simulink library "snn_champions_lib"  (R2026a)
settings: Solver=VariableStepAuto
(part 5 of 24)

== matlab function snn_champions_lib/Donatello_ACC_IIDM_M/IIDM_CTRL ==
  data: s input; accel output; v input; dv input; v_l input
function accel = IIDM_CTRL(s, v, dv, v_l)
%#codegen
% SP4-M-FSM #2a - Donatello + ACC-IIDM con le 5 divisioni sequenziate su UNA divide() condivisa.
%  UNA sola chiamata a fsm_div in tutto il sorgente, dentro uno stato della FSM -> HDL Coder genera
%  UN divisore, riusato in 5 cicli. `kdiv` e' STATO, non indice di loop: un `for k=1:5` verrebbe
%  SROTOLATO dal codegen -> 5 divisori (giusto nel model acc_iidm_fsm, LETALE qui).
%  Nessun blocco accanto alla chart -> niente conversione MATLAB-to-dataflow -> tanh fixed NATIVA:
%  e' cio' che ha ucciso #1 (blocco Divide esterno) -- HDL_PHASE §9.
%  La matematica NON e' qui: sta in iidm_prep/iidm_nd/iidm_use/iidm_final, le STESSE del model
%  acc_iidm_fsm (G2: dmax=0 su 60000 control-step). Qui c'e' solo l'orchestrazione.
%
%  UNO STADIO PER CICLO (misurato: la prima versione faceva decode+prep in un ciclo e nd+div+use in
%  un altro -> path critico 701 livelli, Fmax 2,85 MHz, timing non chiuso). Il time-mux della FSM
%  taglia l'AREA; l'Fmax la da' il REGISTRO fra gli stadi: ogni fase fa UNA cosa e latcha il
%  risultato, cosi' il path piu' lungo e' al massimo quello di uno stadio (la divisione).
  Tt = snn_types('fixed', 13);
  Ta = acc_types('fixed');
  xn = local_normalize(s, v, dv, v_l, Tt);
  % alf/vlp (stato del filtro OU) vivono QUI, nel top-level: HDL Coder vieta i persistent in una
  % funzione non-entry-point chiamata in un condizionale, e iidm_prep e' chiamata in due rami.
  persistent pv xprev started acc phase kdiv st alf vlp rawl numl denl ql thl dA dR dQ dB dsq dkbit dns sX sR sQ sk sabv dkv dfrv blv ouv dsv acbl dadj qaf qbf ds0 ddel
  if isempty(started)
    pv = fi(zeros(5,1), 1, 21, 13);
    xprev = xn; started = true;
    acc = cast(0, 'like', Ta.out);
    phase = uint8(0); kdiv = uint8(1);
    alf = cast(0, 'like', Ta.acc); vlp = cast(v_l, 'like', Ta.st);
    % [R9] ouv: il TIPO viene dall'espressione dentro iidm_prep_a, non da una dichiarazione
    [ouv, alf, vlp] = iidm_prep_a(v_l, true, alf, vlp);
    % `pv(:)` (fi) e NON zeros(5,1) (double): due tipi diversi di `p` darebbero DUE specializzazioni
    % di iidm_prep, in silenzio.
    % [R2] stato della radice sequenziale: X radicando (consumato 2 bit per passo), R resto,
    % Q radice parziale, sk contatore di passi (STATO: un for verrebbe srotolato -> 10 radici).
    sX = fi(0, 0, sqrt_seq_nb()*2, 0); sR = fi(0, 0, sqrt_seq_nb()+2, 0);
    sQ = fi(0, 0, sqrt_seq_nb(), 0);   sk = uint8(0);
    % Il TIPO di sabv lo da' sqrt_seq_fin, non una costante scritta a mano: una sola definizione
    % (su un argomento nullo e' un reinterpretcast di una costante -> zero hardware).
    sabv = sqrt_seq_fin(sQ);
    % [R4] stato fra le due meta' del decode. I tipi sono quelli delle uscite di decode_a: se
    % sbagliassi, il codegen fallisce RUMOROSAMENTE (conflitto di tipo su persistent), non in silenzio.
    dkv = zeros(5,1,'int32'); dfrv = fi(zeros(5,1), 1, 16, 14);
    dsv = fi(zeros(5,1), 1, 16, 14);   % tipo Ts, lo stesso dichiarato in decode_b
    ds0 = fi(zeros(5,1), 1, 16, 14); ddel = fi(zeros(5,1), 1, 16, 14);   % [R17] tipo Ts
    dadj = fi(zeros(5,1), 1, 18, 13);   % tipo Tadj, lo stesso dichiarato in decode_a1
    [qaf, qbf] = iidm_ab(pv(:));   % [R14] tipi dedotti da iidm_ab (T.par)
    [st, alf, vlp] = iidm_prep(s, v, dv, v_l, pv(:), true, alf, vlp, sabv);
    rawl = fi(zeros(5,1), 1, 21, 13);   % latch del readout SNN: spezza il path SNN -> decode
    numl = cast(0, 'like', Ta.acc); denl = cast(1, 'like', Ta.acc); ql = cast(0, 'like', Ta.acc);
    % [IIDM #2] stato della ricorrenza: A dividendo residuo, R resto, Q quoziente, B divisore,
    % dsq segno, dkbit contatore di bit (STATO: un for verrebbe srotolato -> 27 divisori).
    dA = fi(0, 0, div_seq_nb(), 0); dQ = fi(0, 0, div_seq_nb(), 0);
    dR = fi(0, 0, 20, 0); dB = fi(0, 0, 20, 0);
    dsq = false; dkbit = uint8(0); dns = int8(0);
    % thl col TIPO NATIVO di tanh (NON cast a Ta.acc: butterebbe i bit frazionari del tanh prima
    % del prodotto con bf -> bug §2.1). Il tipo lo da' tanh stesso su un argomento di tipo Ta.acc.
    thl = tanh(cast(0, 'like', Ta.acc));
    % [R6] blv DOPO st e thl: il suo TIPO viene dall'espressione, non da una dichiarazione a mano
    % (cosi' non posso sbagliare la larghezza). Ordine obbligato: iidm_final_a li usa entrambi.
    blv = iidm_final_a(st, thl);
    acbl = iidm_final_b(st, blv);   % stesso principio: TIPO dedotto dall'espressione
    go = true;
  else
    go = any(xn ~= xprev);             % edge-triggered: 1 campione = 1 inferenza (§3.1.4)
  end
  xprev = xn;
  [raw, valid] = snn_b2_fsm(xn, go);
  if phase == 1                        % [R4] DECODE-A: indice di tabella + frazione
    dadj = decode_a1(rawl);
    phase = uint8(20);
  elseif phase == 20                   % [R12] DECODE-A2: scala, indice di tabella e frazione
    [dkv, dfrv] = decode_a2(dadj, 64);
    phase = uint8(12);
  elseif phase == 12                   % [R4] DECODE-B: interpolazione -> i 5 parametri IIDM
    [ds0, ddel] = decode_b1(dkv, 64);
    phase = uint8(23);
  elseif phase == 23                   % [R17] DECODE-B2: interpolazione lineare s0 + frac*del
    dsv = decode_b2(ds0, ddel, dfrv);
    phase = uint8(18);
  elseif phase == 18                   % [R10] DECODE-C: scalatura finale -> i 5 parametri
    pv = decode_c(dsv);
    phase = uint8(10);
  elseif phase == 10                   % [R2] SQRT-INIT: il radicando af*bf entra nella ricorrenza
    [qaf, qbf] = iidm_ab(pv(:));
    phase = uint8(21);
  elseif phase == 21                   % [R14] SQRT-PRE: il prodotto af*bf entra nella ricorrenza
    sX = sqrt_seq_setup(iidm_sabx_mul(qaf, qbf));
    sR(:) = 0; sQ(:) = 0; sk = uint8(sqrt_seq_nb());
    phase = uint8(11);
  elseif phase == 11                   % [R2] SQRT-STEP: 2 bit di radicando per ciclo, 10 cicli
    [sX, sR, sQ] = sqrt_seq_step(sX, sR, sQ);
    sk = sk - uint8(1);
    if sk == uint8(0)
      sabv = sqrt_seq_fin(sQ);         % SQRT-FIN: tipizzazione finale (reinterpretcast, zero HW)
      phase = uint8(2);
    end
  elseif phase == 2                    % PREP (un ciclo a se': guardie, filtro OU; la sqrt arriva fatta)
    [ouv, alf, vlp] = iidm_prep_a(v_l, false, alf, vlp);   % 1 volta per control-step (§5)
    phase = uint8(17);
  elseif phase == 17                   % [R9] OU-B: il passo esponenziale del filtro
    alf = iidm_prep_a2(ouv, alf);
    phase = uint8(16);
  elseif phase == 16                   % [R8] PREP-B: cast + costruzione dello struct
    st = iidm_prep_b(s, v, dv, v_l, pv(:), alf, sabv);
    kdiv = uint8(1); phase = uint8(3);
  elseif phase == 3                    % ND: SOLO gli operandi della divisione k
    [numl, denl] = iidm_nd(kdiv, st);
    phase = uint8(4);
  elseif phase == 4                    % DIV-INIT: magnitudini + segno (div_seq_setup)
    [dA, dB, dsq] = div_seq_setup(numl, denl);
    dR(:) = 0; dQ(:) = 0; dkbit = uint8(div_seq_nb());
    dns = int8(0);
    if numl > 0
      dns = int8(1);
    elseif numl < 0
      dns = int8(-1);
    end
    phase = uint8(8);
  elseif phase == 8                    % DIV-STEP: UN bit di quoziente per ciclo
    [dA, dR, dQ] = div_seq_step(dA, dR, dQ, dB);
    dkbit = dkbit - uint8(1);
    if dkbit == uint8(0)
      phase = uint8(9);
    end
  elseif phase == 9                    % DIV-FIN: segno + saturazione -> ql
    ql(:) = div_seq_fin(dQ, dsq, dB == 0, dns);
    phase = uint8(5);
  elseif phase == 5                    % [R5] USE-A: SOLO i quadrati (k=2: q^2, k=3: z e z^2)
    st = iidm_use_a(kdiv, ql, st);
    phase = uint8(15);
  elseif phase == 15                   % [R7] USE-M: il secondo quadrato (k=2: uu^2)
    st = iidm_use_m(kdiv, st);
    phase = uint8(22);
  elseif phase == 22                   % [R16] USE-M2: secondo quadrato (k=2) / sottrazione (k=3)
    st = iidm_use_m2(kdiv, st);
    phase = uint8(13);
  elseif phase == 13                   % [R5] USE-B: prodotti e selezioni
    st = iidm_use_b(kdiv, ql, st);
    if kdiv >= 5
      phase = uint8(6);
    else
      kdiv = kdiv + 1; phase = uint8(3);
    end
  elseif phase == 6                    % TANH: stadio a se' -- era il PATH CRITICO (237 liv, 7,35 MHz)
    thl(:) = iidm_tanh(st);
    phase = uint8(7);
  elseif phase == 7                    % [R6] FINAL-A: a_cah + bf*th (il prodotto col tanh)
    blv = iidm_final_a(st, thl);
    phase = uint8(14);
  elseif phase == 14                   % [R6] FINAL-B: blend + clamp -> accel (tenuta fino al prossimo)
    acbl = iidm_final_b(st, blv);
    phase = uint8(19);
  elseif phase == 19                   % [R11] FINAL-C: cast + selezione ACC + clamp -> accel
    acc = iidm_final_c(st, acbl);
    phase = uint8(0);
  end
  if valid                             % [2d R1] latch DOPO la catena: rawl e' un vero registro
    rawl(:) = raw;                     %   -> readout (pR_idx->raw) e decode (rawl->pv) DISACCOPPIATI
    phase = uint8(1);
  end
  accel = acc;
end

function xn = local_normalize(s, v, dv, v_l, T)
%LOCAL_NORMALIZE  fisico -> xn (fixed). Nel deployato la normalize gira in SW float e all'HDL
%  arriva gia' xn (HDL_PHASE §3.1); qui sta nel blocco per avere I/O fisico.
%  RECIPROCI a Q?.30 (NON Q?.20): verificato che con Q?.20 l'arrotondamento di xn devia di 1 LSB
%  dal path float ~1 volta su 25 step -> uno spike flippa -> i params divergono. Con Q?.30 e
%  ingressi con >=20 bit frazionari, xn e' IDENTICO al riferimento float (0 diff).
  invS   = fi(0.0066666666666666671, 1, 34, 30);
  invV   = fi(0.025000000000000001, 1, 34, 30);
  inv2DV = fi(0.025000000000000001, 1, 34, 30);
  invVL  = fi(0.025000000000000001, 1, 34, 30);
  DVc    = fi(20, 1, 24, 13);   % 24-13-1 = 10 bit interi: DV=20 ci sta
                                     % (con Q5.13/18bit saturerebbe a ~16 -> clamp sbagliato)
  d = dv;                            % clamp a +-DV. NB: d(:) = ... per NON cambiare il tipo di d
  if d >  DVc, d(:) =  DVc; end      %     (codegen: una variabile non puo' cambiare tipo, HDL_PHASE §9)
  if d < -DVc, d(:) = -DVc; end
  xn = cast(zeros(4,1), 'like', T.V);
  xn(1) = cast(s * invS, 'like', T.V);
  xn(2) = cast(v * invV, 'like', T.V);
  xn(3) = cast((d + DVc) * inv2DV, 'like', T.V);
  xn(4) = cast(v_l * invVL, 'like', T.V);
end

% ====================================================================================
% Funzioni locali INLINATE dai sorgenti veri (build_hdl_variants le legge a build-time).
% Le funzioni locali hanno precedenza sul path => il blocco e' SELF-CONTAINED.
% NON modificarle qui: si rigenerano con build_hdl_variants.
% ====================================================================================

function W = b2_rom_active() %#codegen
%B2_ROM_ACTIVE  Pesi del champion attivo (baked). GENERATO da gen_b2_rom('Donatello').
  W.fc = fi([1 1 -0.25 1;0.125 0.5 -0.0625 1;1 -1 1 0.125;1 0.125 0.5 -0.125;1 0.5 -0.0625 0.5;-0.0625 0.25 0 1;0 0.5 0.5 0.25;1 -0.25 2 -0.0625;1 0.125 -0.25 0.5;0.25 1 0.125 -0.25;0.25 -0.25 0.5 1;0.5 -0.5 0.5 0.25;1 0.25 -0.125 0.5;-1 1 0.25 0.5;1 0.5 1 -0.25;0.5 -0.25 0.5 0.0625;0.25 -0.25 1 -0.5;-0.5 -0.5 1 0.25;2 0 -0.25 0;-0.5 0.5 0.5 1;-0.125 -0.25 1 0;1 0.125 1 -0.5;-0.0625 1 0.5 0.125;1 1 -0.25 -0.125;2 0.5 0.5 -0.25;-0.125 0.5 0.25 -0.25;1 0.125 -0.0625 0.25;-0.5 -0.25 1 0.5;1 -0.125 0.125 0.5;1 -0.0625 0.5 0.25;1 0.5 1 0.125;0.125 0.25 0.5 0], 1, 16, 13);
  W.U = fi([0 0 -0.0625 -0.0625 -0.0625 0 0 0 -0.0625 0 0 0 0.0625 0 -0.125 0;-0.0625 0 -0.0625 0 0 0 0 0 0 0 -0.0625 0 0 0.0625 0 0;0.0625 -0.0625 -0.0625 0 -0.0625 -0.0625 0 0 0.0625 0 0.0625 0 0 0 0 0;0.0625 -0.0625 0 0 0 0 -0.0625 0 0 -0.0625 0.0625 -0.0625 0 -0.0625 0 -0.0625;0.0625 -0.0625 0 0 0 0 0.0625 0 0 0 0 -0.0625 0.0625 0 -0.0625 0;0 0.0625 0.0625 -0.0625 0.0625 0 0 0 0.0625 0.0625 0 0.0625 0 0 0 0;-0.0625 0.0625 0.0625 -0.0625 0 0 -0.0625 0.0625 0.0625 0.0625 0 0 -0.0625 0 0 0.0625;0 0 0.0625 0.0625 0 0 0 0 -0.0625 -0.0625 0 0 0 0 -0.0625 0;0 0 0 0 0.0625 -0.0625 0 0 -0.0625 -0.0625 -0.0625 0 0 0 0.0625 0;0 0 0 0 0.0625 0 0 0 0.0625 -0.0625 0 0.0625 0 0 0 0.0625;0 0 0 0 0 0 0 -0.0625 0 0 -0.0625 0 0 0 0 0.0625;0 0.0625 0 0.0625 0 0 0 0.0625 0 -0.0625 0 -0.0625 0.0625 0 0 0;-0.0625 0.0625 0 0 0 0 -0.0625 0 0.0625 0 -0.0625 0 0 0 0 0.125;0 0 0 0 0 0.0625 -0.0625 -0.0625 0 0.0625 0 0 0.0625 0.0625 0.0625 0;0.0625 0.0625 -0.0625 0 0 -0.0625 -0.0625 0 0 0 -0.0625 0 -0.0625 0 0 0;0.0625 0 0 0 -0.0625 -0.0625 -0.0625 0.0625 -0.0625 -0.0625 0 0.0625 0 0 0 0.0625;-0.0625 0 0 0 0.125 0.0625 -0.0625 -0.0625 0 0 0 0 -0.0625 0 -0.0625 0;0.0625 -0.0625 0 0.0625 0 -0.125 0 -0.0625 0 0 0.0625 -0.0625 0.0625 0 -0.0625 -0.0625;-0.0625 0 -0.0625 0.0625 -0.0625 0 -0.0625 0.0625 0.0625 -0.0625 0 0 -0.0625 0 0 -0.0625;0.0625 0.125 0 -0.0625 0 0 0 0 0.0625 0 0.0625 0.0625 0 0 -0.0625 0;0 -0.0625 0 0 -0.125 -0.0625 0 0.0625 -0.0625 -0.0625 0.0625 0 0.0625 -0.0625 -0.0625 -0.0625;0 0 0 0 -0.0625 0 0.0625 -0.0625 0 -0.0625 0.0625 0 0.0625 0 0 0;-0.0625 0.125 0 0 0 -0.0625 0 0 -0.0625 0.0625 0 0 0 0 0.0625 0;0 0 0 0 0 0 0 0 -0.0625 0 0.0625 0.125 0 0.0625 0 0.0625;0 -0.0625 0.0625 0 0 -0.0625 0 0 -0.0625 0 0 0.0625 0.0625 0 0 0;-0.0625 0 0 -0.125 0.0625 0.0625 0 0 0 0.0625 -0.0625 0.0625 -0.0625 0.0625 0.0625 0;0.0625 -0.0625 0 0 0 0 0.0625 0 -0.0625 0 0 0 0 0 0 0.0625;0 0 0 0.125 0 0 0 0.0625 -0.0625 0 0.0625 -0.0625 0 0.0625 0 0;0 0.0625 0.0625 0 0 0.0625 -0.0625 0 0 0.0625 0 0 -0.0625 0 0.0625 0.125;0 0.0625 0.0625 0.0625 0.0625 0.0625 0 0 0 0.0625 -0.0625 0.0625 -0.0625 0 0 0;0 0 0.0625 0 0 0.0625 -0.0625 -0.0625 0.0625 0.0625 -0.0625 0.125 0.0625 0 0 0;0 0 -0.0625 0.0625 0.0625 0 0 0.125 0 0.0625 0.0625 0.0625 0 -0.0625 0.0625 0], 1, 16, 13);
  W.Vr = fi([0 -0.125 -0.0625 -0.0625 0 0 -0.0625 -0.0625 0 -0.0625 -0.0625 0 0 0 -0.0625 -0.0625 0 0 0.0625 0 0 -0.125 0 0.0625 0 0 -0.0625 0 0 0 0 0;0.0625 0.0625 0 0 0 0 0.0625 0 0 0.0625 0.0625 0 0 0 0 0.0625 0 -0.0625 0 0.0625 0 0 0.0625 0 0.0625 0 0 0.125 -0.0625 0.125 0 0;0 0.0625 0 0.0625 0 0 -0.0625 0 0 0 0 0 0 0.0625 0 0 0.0625 0 0.0625 0 0 0.0625 0.0625 0 -0.0625 -0.0625 0 0 0 0.0625 0 0.0625;0 -0.0625 -0.0625 0 0 0 0 -0.0625 0 0 0.0625 0.0625 0 0 0 0.0625 0.0625 0 -0.0625 -0.0625 -0.0625 -0.0625 0.0625 0 0 0 0 0 0.0625 -0.0625 -0.0625 0;0 0 0.0625 0 -0.0625 0.0625 0.0625 0.0625 0 0 0.0625 0 0.0625 0.0625 0.0625 0 0.0625 0 0.0625 0 0.0625 0 0 0.0625 0.0625 0 0.125 0 0 0.0625 0.0625 0;0 0.0625 -0.125 0 0 0 0 0 0 -0.0625 -0.0625 0 0 0.0625 0.125 0.0625 0 0.0625 -0.0625 0.0625 0.0625 0 0.0625 -0.0625 0 -0.0625 0 0 0 0.0625 0 0;0 -0.0625 -0.0625 0 0 -0.0625 0 -0.0625 0 0 -0.0625 -0.0625 -0.0625 0.0625 -0.0625 0 0 -0.0625 0.0625 -0.125 -0.0625 0 -0.0625 -0.0625 -0.0625 0 0 -0.125 -0.0625 0 0 -0.0625;0 0 -0.0625 -0.0625 0.0625 0 -0.0625 0 -0.0625 0 0.0625 -0.0625 0.0625 0.0625 0.0625 0 0 0 0 -0.0625 0 -0.0625 0 0 0 0 -0.0625 -0.0625 0 0 0 0;-0.0625 0.0625 0 0.0625 0 0.0625 -0.0625 0 0.0625 0 0.0625 0 0 0.0625 0 0 0 0 0.0625 -0.0625 0.0625 0 0.0625 0 0 0.125 0.0625 0.0625 0.0625 0.0625 0 0;0.0625 0.0625 0 0.0625 0.0625 0.0625 0.0625 0.0625 0.0625 0 0.0625 0 0.0625 0.0625 0 -0.0625 0.0625 0 0.0625 0.0625 0 0.0625 0.0625 0 0.0625 0.0625 0 0 0 0 0 0;0 -0.0625 -0.0625 0 -0.0625 0 0 0 0 0 -0.0625 -0.125 -0.0625 -0.0625 0 -0.0625 -0.0625 0 0 -0.0625 -0.0625 0 0 0 0 -0.0625 0 -0.0625 0 0 -0.0625 0;0 0 0 0.0625 0 0 0.0625 0 0 0 0 0 0.0625 0 0 0.125 -0.0625 0 0.0625 0.0625 0 0 0.0625 0.0625 0 0.0625 0.0625 0 0 0 0 0;-0.0625 0 0 0 0.0625 0.0625 0 -0.0625 -0.0625 -0.0625 -0.0625 0 0 -0.0625 0 -0.0625 0 0 0 -0.0625 0 -0.0625 0 0 -0.0625 -0.0625 0 0 -0.0625 0 0.0625 0;0.0625 0 0 0.0625 0 0 0 -0.0625 0 0.0625 0 -0.0625 0 0.0625 0.0625 0 0.0625 0.0625 0 0.0625 0 0 0 0.0625 0.0625 0 0 0.125 0 0 0.0625 -0.0625;0.0625 0 0 0.0625 0 0.0625 0 0 0 0.0625 -0.0625 -0.0625 0 0.125 0 0 0 0 -0.0625 0 0.0625 0 0.0625 -0.0625 0.0625 0 0 0 0 0 0.0625 0;0 0 0 0.0625 0 0.0625 0 0.0625 0 0 0.0625 0.0625 0 0 0 0.0625 -0.0625 0 0.0625 0.0625 0.0625 0 0 0.0625 0.125 0 0 0 0 0 0.0625 0], 1, 19, 13);
  W.Wout = fi([-0.25 -0.125 -0.0625 -0.25 -0.25 0.25 0.25 -0.5 0.125 0.125 0.5 0.25 0.5 -0.125 0.25 0.25 -0.5 -0.25 0.0625 0.25 -0.25 0.0625 0 0.125 -0.25 0.25 0.25 -0.25 0 0 0.125 0.5;0.125 -0.125 0.25 -0.25 -0.125 0 -0.25 0 -0.25 0 0 0 -0.5 -0.5 0.125 0.25 -0.5 0.125 -0.25 0 0.25 0.25 -0.25 0.25 0.25 0 0.5 -0.25 -0.125 -0.25 0.0625 0.0625;0 -0.25 -0.25 0.125 -0.5 -0.0625 0 -0.125 0.125 0 0.25 -0.0625 -0.25 0.25 0.0625 -0.125 -0.25 0.125 -0.5 0.125 0.25 -0.5 -0.25 -0.25 0.25 0.25 0 0.5 -0.125 -0.5 0.125 0.125;0.5 0 0.25 0.25 0.25 -0.5 0.25 -0.25 0.5 0 -0.5 0.125 -0.0625 -0.5 -0.125 0.0625 0.25 -0.125 0.25 0.0625 0 0.0625 -0.25 -0.25 -0.125 -0.5 -0.25 0 -0.25 -0.125 -0.0625 -0.0625;-0.25 0 -0.0625 0.0625 0 -0.25 -0.125 -0.0625 -0.25 0 -0.0625 0.125 0.0625 0.25 -0.0625 -0.25 0.125 -0.25 -0.0625 -0.125 -0.25 -0.125 0.25 0.25 0.0625 0.25 -0.5 0.0625 0.25 0.25 -0.25 0.125], 1, 16, 13);
  W.bth = fi([1.4830578565597534;1.4914478063583374;1.4758200645446777;1.4738426208496094;1.4738566875457764;1.5251744985580444;1.5266332626342773;1.4767427444458008;1.4758551120758057;1.5250141620635986;1.5258395671844482;1.5129754543304443;1.5257152318954468;1.5249043703079224;1.5155367851257324;1.5183815956115723;1.5177655220031738;1.4894863367080688;1.4749715328216553;1.5253423452377319;1.4770052433013916;1.4827579259872437;1.5239431858062744;1.5230189561843872;1.4776254892349243;1.5125672817230225;1.5243701934814453;1.4934873580932617;1.5239229202270508;1.5202276706695557;1.5248651504516602;1.5149734020233154], 1, 19, 13);
  W.tj = fi([0.49987733364105225;0.49987733364105225;0.49987733364105225;0.49987733364105225;0.49987733364105225;0.49987733364105225;0.49987733364105225;0.49987733364105225;0.49987733364105225;0.49987733364105225;0.49987733364105225;0.49987733364105225;0.49987733364105225;0.49987733364105225;0.49987733364105225;0.49987733364105225;0.49987733364105225;0.49987733364105225;0.49987733364105225;0.49987733364105225;0.49987733364105225;0.49987733364105225;0.49987733364105225;0.49987733364105225;0.49987733364105225;0.49987733364105225;0.49987733364105225;0.49987733364105225;0.49987733364105225;0.49987733364105225;0.49987733364105225;0.49987733364105225], 1, 19, 13);
  W.delays = [3 5 1 2;2 4 4 4;2 4 0 4;5 0 5 5;1 2 2 2;4 1 4 2;0 4 0 1;0 1 0 1;2 2 1 3;1 2 5 2;0 5 1 2;0 5 3 1;2 0 0 4;2 2 3 4;4 4 5 0;4 5 0 2;0 4 4 3;5 5 4 2;4 5 4 2;3 0 3 1;3 2 0 4;0 4 2 0;5 4 5 2;4 4 3 3;5 3 4 5;2 2 3 1;3 3 5 3;1 3 0 3;1 0 3 2;2 3 4 4;2 4 5 0;1 2 4 0];
  W.sh = 3;
  W.invS = fi(0.0066666666666666671, 1, 24, 20);
  W.invV = fi(0.025000000000000001, 1, 24, 20);
  W.invVL = fi(0.025000000000000001, 1, 24, 20);
  W.inv2DV = fi(0.025000000000000001, 1, 24, 20);
  W.DV = fi(20, 1, 20, 13);
end


function T = snn_types(dt, nfrac)
%SNN_TYPES Prototipi di tipo per il core type-parametrizzato.
%  dt = 'double' (parita' vs golden) | 'fixed' (HDL, Qm.n).
%  nfrac (opz., default 5) = bit frazionari del path fixed; i bit INTERI restano
%  fissi (range invariato), varia solo la risoluzione -> per tarare i word-length
%  col ginocchio errore/risorse (run_fixed_sweep). nfrac=5 == config storica.
  if nargin < 2, nfrac = 5; end
  switch dt
    case 'double'
      z = double([]);
      T = struct('V', z, 'fatigue', z, 'acc', z, 'accw', z, 'raw', z, 'w', z);
    case 'fixed'
      f = nfrac;
      T = struct( ...
        'V',       fi([], true, 6 + f, f), ...    % Q5.f  (int 5)
        'fatigue', fi([], true, 4 + f, f), ...    % Q3.f  (int 3)
        'acc',     fi([], true, 6 + f, f), ...    % accumulatore I_input Q5.f (int 5: un tap di delay arriva a ~8)
        'accw',    fi([], true, 13 + f, f + 4), ...% accumulatore LARGO Q8.(f+4): +4 frac per shift po2 esatti
        'raw',     fi([], true, 8 + f, f), ...    % readout LI Q7.f (int 7)
        'w',       fi([], true, 3 + f, f));       % pesi po2 Q2.f (esatti per f>=5)
    otherwise
      error('snn_types:dt', 'dt deve essere ''double'' o ''fixed''');
  end
end


function [raw, valid] = snn_b2_fsm(xn, start) %#codegen
%SNN_B2_FSM  [B2] SNN Donatello time-multiplexato (1 neurone/clock) con hdl.RAM.
%  Mirror BIT-EXACT dell'aritmetica di snn_core, serializzato: V/fatigue in hdl.RAM,
%  pesi in ROM (coder.const), pipeline a 2 stadi per la latenza RAM (read->compute->write,
%  1 sola chiamata RAM/ciclo). Streaming: start=1 -> nuova control-step; valid=1 -> raw pronto.
  W = coder.const(b2_rom_active());
  T = snn_types('fixed', 13);
  hidden = 32; nt = 10; rnk = coder.const(size(W.U, 2)); out = 5; sh = W.sh;

  persistent Vram fatram xbuf xnreg t_lr t_lr_nxt V_LI wacc ...
             tickc rc written phase ...
             pR_valid pR_idx pCx_valid pCx_idx pCx_xsel pCx_Vread pCx_fat ...
             pCm_valid pCm_idx pCm_Iip pCm_recip pCm_Vread pCm_fat ...
             pCa_valid pCa_idx pCa_reci pCa_Ii pCa_Vread pCa_fat ...
             pC1_valid pC1_idx pC1_Ii pC1_reci pC1_Vread pC1_fat ...
             pC2i_valid pC2i_idx pC2i_Vi pC2i_eth pC2i_fat ...
             pC2a_valid pC2a_idx pC2a_nCV pC2a_sib pC2a_fat ...
             pC_valid pC_idx pC_V pC_fat rawreg inited
  if isempty(inited)
    Vram   = hdl.RAM('RAMType', 'Dual port');
    fatram = hdl.RAM('RAMType', 'Dual port');
    xbuf   = cast(zeros(4, 6), 'like', T.V);
    xnreg  = cast(zeros(4, 1), 'like', T.V);
    t_lr     = cast(zeros(rnk, 1), 'like', T.acc);
    t_lr_nxt = cast(zeros(rnk, 1), 'like', T.acc);
    V_LI = cast(zeros(out, 1), 'like', T.raw);
    wacc = cast(zeros(out, 1), 'like', T.raw);
    tickc = uint8(0); rc = uint8(0); written = uint8(0); phase = uint8(0);
    pR_valid = false; pR_idx = uint8(0);
    pCx_valid = false; pCx_idx = uint8(0);
    pCx_xsel = cast(zeros(4, 1), 'like', T.V);
    pCx_Vread = cast(0, 'like', T.V); pCx_fat = cast(0, 'like', T.fatigue);
    pCm_valid = false; pCm_idx = uint8(0);
    pCm_Iip = cast(zeros(4, 1), 'like', T.accw); pCm_recip = cast(zeros(rnk, 1), 'like', T.accw);
    pCm_Vread = cast(0, 'like', T.V); pCm_fat = cast(0, 'like', T.fatigue);
    pCa_valid = false; pCa_idx = uint8(0);
    pCa_reci = cast(zeros(rnk/4, 1), 'like', T.accw);   % rnk/4 somme parziali (dopo 2 livelli d'albero)
    pCa_Ii = cast(0, 'like', T.accw);
    pCa_Vread = cast(0, 'like', T.V); pCa_fat = cast(0, 'like', T.fatigue);
    pC1_valid = false; pC1_idx = uint8(0);
    pC1_Ii = cast(0, 'like', T.accw); pC1_reci = cast(0, 'like', T.accw);
    pC1_Vread = cast(0, 'like', T.V); pC1_fat = cast(0, 'like', T.fatigue);
    % [2d R8] prototipi dei tipi LARGHI di Vi/eth (l'addizione fixed li allarga oltre T.V): servono per
    % registrarli fra C2i (Vi/eth) e C2a (soglia/nC_V) senza conflitto di tipo in codegen.
    zV = cast(0, 'like', T.V); zA = cast(0, 'like', T.accw); zF = cast(0, 'like', T.fatigue);
    Vi0  = cast(zV - bitsra(zV, sh), 'like', T.V) + (zA + zA);
    eth0 = cast(zV, 'like', T.V) + cast(max(zF, zF), 'like', T.V);
    pC2i_valid = false; pC2i_idx = uint8(0);
    pC2i_Vi = cast(0, 'like', Vi0); pC2i_eth = cast(0, 'like', eth0);
    pC2i_fat = cast(0, 'like', T.fatigue);
    pC2a_valid = false; pC2a_idx = uint8(0);
    pC2a_nCV = cast(0, 'like', T.V); pC2a_sib = cast(0, 'like', T.V);
    pC2a_fat = cast(0, 'like', T.fatigue);
    pC_valid = false; pC_idx = uint8(0);
    pC_V = cast(0, 'like', T.V); pC_fat = cast(0, 'like', T.fatigue);
    rawreg = cast(zeros(out, 1), 'like', T.raw);
    inited = true;
  end

  valid = false;
  raw = rawreg;

  % ---------- helper x_buf: shift + inserimento xnreg (inizio tick) ----------
  % (fatto inline dove serve)

  if phase == uint8(0)
    % IDLE: su start latcha xn, fa lo shift del tick 0, avvia la pipeline
    if start
      xnreg = xn;
      xbuf(:, 2:6) = xbuf(:, 1:5); xbuf(:, 1) = xnreg;   % tick 0 shift+insert
      tickc = uint8(0); rc = uint8(0); written = uint8(0);
      wacc = cast(zeros(out, 1), 'like', T.raw);
      pR_valid = false; pC_valid = false;
      phase = uint8(1);
    end
    % passo RAM idle (mantiene coerenza)
    [~, ~] = Vram(cast(0,'like',T.V), uint8(0), false, uint8(0));
    [~, ~] = fatram(cast(0,'like',T.fatigue), uint8(0), false, uint8(0));
    return;
  end

  % ---------- FASE 1: RUN (pipeline 2-stadi, 1 chiamata RAM/ciclo) ----------
  % indirizzo di lettura per questo ciclo (neurone rc, se ancora da leggere)
  if rc < uint8(hidden), rdAddr = rc; else, rdAddr = uint8(0); end

  % UNA chiamata RAM: scrive il risultato dello stadio C (pC), legge rdAddr
  [~, Vread]   = Vram(pC_V,   pC_idx, pC_valid, rdAddr);
  [~, fatread] = fatram(pC_fat, pC_idx, pC_valid, rdAddr);
  if pC_valid
    written = written + uint8(1);
  end

  % --- STADIO Cx (mux xbuf: seleziona i 4 ingressi ritardati): dal neurone pR ---
  % [2d R9] separo il mux a indice variabile xbuf(j,col) dal DSP mult: Cx registra i 4 valori selezionati
  % (xsel), Cm fa solo i moltiplicatori dai valori registrati -> il mult (~4,6ns) resta l'unico op del suo path.
  nCx_valid = false; nCx_idx = uint8(0);
  nCx_xsel = cast(zeros(4, 1), 'like', T.V);
  nCx_Vread = cast(0, 'like', T.V); nCx_fat = cast(0, 'like', T.fatigue);
  if pR_valid
    i = double(pR_idx) + 1;
    for j = 1:4
      col = double(W.delays(i, j)) + 1;
      nCx_xsel(j) = xbuf(j, col);
    end
    nCx_Vread = Vread; nCx_fat = fatread;
    nCx_valid = true; nCx_idx = pR_idx;
  end

  % --- STADIO Cm (MAC: 16 prodotti reci + 4 prodotti Ii, REGISTRATI): dagli ingressi mux registrati pCx ---
  % [2d R6] isolo i moltiplicatori: Cm calcola e REGISTRA i prodotti (uscite DSP), Ca fa gli alberi dai
  % prodotti registrati -> il DSP mult (~4,6ns) esce dal path degli alberi (mappato sul registro P del DSP48).
  % Bit-exact: stessi prodotti, solo registrati.
  nCm_valid = false; nCm_idx = uint8(0);
  nCm_Iip = cast(zeros(4, 1), 'like', T.accw);
  nCm_recip = cast(zeros(rnk, 1), 'like', T.accw);
  nCm_Vread = cast(0, 'like', T.V); nCm_fat = cast(0, 'like', T.fatigue);
  if pCx_valid
    i = double(pCx_idx) + 1;
    for j = 1:4
      nCm_Iip(j) = cast(cast(W.fc(i, j), 'like', T.w) * pCx_xsel(j), 'like', T.accw);
    end
    for r = 1:rnk
      nCm_recip(r) = cast(cast(W.U(i, r), 'like', T.w) * t_lr(r), 'like', T.accw);
    end
    nCm_Vread = pCx_Vread; nCm_fat = pCx_fat;
    nCm_valid = true; nCm_idx = pCx_idx;
  end

  % --- STADIO Ca (alberi: Ii 4->1, reci L1-L2 16->4): dai prodotti registrati pCm ---
  kmid = coder.const(rnk / 4);                    % rnk=16 -> 4 parziali dopo 2 livelli
  nCa_valid = false; nCa_idx = uint8(0);
  nCa_reci = cast(zeros(kmid, 1), 'like', T.accw);
  nCa_Ii = cast(0, 'like', T.accw);
  nCa_Vread = cast(0, 'like', T.V); nCa_fat = cast(0, 'like', T.fatigue);
  if pCm_valid
    % Ii ad albero (4->2->1) dai prodotti registrati
    Ii_p = pCm_Iip;
    Ii_p(1) = cast(Ii_p(1) + Ii_p(2), 'like', T.accw);
    Ii_p(2) = cast(Ii_p(3) + Ii_p(4), 'like', T.accw);
    nCa_Ii  = cast(Ii_p(1) + Ii_p(2), 'like', T.accw);
    % reci: primi 2 livelli d'albero (16->4) dai prodotti registrati
    reci_p = pCm_recip;
    lvsz_a = coder.const(round(rnk ./ 2 .^ (1:2)));   % rnk=16 -> [8 4]
    for lev = 1:2
      for q = 1:lvsz_a(lev)
        reci_p(q) = cast(reci_p(2*q - 1) + reci_p(2*q), 'like', T.accw);
      end
    end
    nCa_reci = reci_p(1:kmid);            % rnk/4 somme parziali (T.accw)
    nCa_Vread = pCm_Vread; nCa_fat = pCm_fat;
    nCa_valid = true; nCa_idx = pCm_idx;
  end

  % --- STADIO C1 (SECONDA meta' dell'albero reci): dal registro pCa ---
  nC1_valid = false; nC1_idx = uint8(0);
  nC1_Ii = cast(0, 'like', T.accw); nC1_reci = cast(0, 'like', T.accw);
  nC1_Vread = cast(0, 'like', T.V); nC1_fat = cast(0, 'like', T.fatigue);
  if pCa_valid
    reci_p2 = pCa_reci;                  % kmid parziali
    lvsz_b = coder.const(round(kmid ./ 2 .^ (1:log2(kmid))));   % kmid=4 -> [2 1]
    for lev = 1:numel(lvsz_b)
      for q = 1:lvsz_b(lev)
        reci_p2(q) = cast(reci_p2(2*q - 1) + reci_p2(2*q), 'like', T.accw);
      end
    end
    nC1_reci = reci_p2(1);
    nC1_Ii = pCa_Ii; nC1_Vread = pCa_Vread; nC1_fat = pCa_fat;   % Vi/soglia -> C2 (tipi larghi restano locali)
    nC1_valid = true; nC1_idx = pCa_idx;
  end

  % --- STADIO C2i (calcola Vi ed eth, tipi larghi 28-bit): dal registro pC1 ---
  % [2d R8] separo Vi/eth (catena di add 28-bit, era il collo in C2a-R7) dalla soglia/nC_V: C2i li produce
  % e REGISTRA (tipi larghi via prototipo Vi0/eth0 in init; init nel corpo via 'like' pC2i_*). Bit-exact.
  nC2i_valid = false; nC2i_idx = uint8(0);
  nC2i_Vi = cast(0, 'like', pC2i_Vi); nC2i_eth = cast(0, 'like', pC2i_eth);
  nC2i_fat = cast(0, 'like', T.fatigue);
  if pC1_valid
    i2 = double(pC1_idx) + 1;
    nC2i_Vi  = cast(pC1_Vread - bitsra(pC1_Vread, sh), 'like', T.V) + (pC1_Ii + pC1_reci);
    nC2i_eth = cast(W.bth(i2), 'like', T.V) + cast(max(pC1_fat, cast(0,'like',T.fatigue)), 'like', T.V);
    nC2i_fat = pC1_fat;
    nC2i_valid = true; nC2i_idx = pC1_idx;
  end

  % --- STADIO C2a (soglia + nC_V + accumulo readout): dal registro pC2i ---
  nC2a_valid = false; nC2a_idx = uint8(0);
  nC2a_nCV = cast(0, 'like', T.V); nC2a_sib = cast(0, 'like', T.V);
  nC2a_fat = cast(0, 'like', T.fatigue);
  if pC2i_valid
    i2  = double(pC2i_idx) + 1;
    si  = pC2i_Vi >= pC2i_eth;
    sib = cast(si, 'like', T.V);
    nC2a_nCV = cast(pC2i_Vi - sib * pC2i_eth, 'like', T.V);
    nC2a_sib = sib; nC2a_fat = pC2i_fat;
    nC2a_valid = true; nC2a_idx = pC2i_idx;
    if si
      for o = 1:out
        wacc(o) = cast(wacc(o) + W.Wout(o, i2), 'like', T.raw);
      end
      for r = 1:rnk
        t_lr_nxt(r) = cast(t_lr_nxt(r) + cast(W.Vr(r, i2), 'like', T.acc), 'like', T.acc);
      end
    end
  end

  % --- STADIO C2b (nC_fat = leaky(fat) + sib*tj): dal registro pC2a; nC_V passa attraverso ---
  nC_valid = false; nC_idx = uint8(0);
  nC_V = cast(0, 'like', T.V); nC_fat = cast(0, 'like', T.fatigue);
  if pC2a_valid
    i3 = double(pC2a_idx) + 1;
    nC_fat = cast(cast(pC2a_fat - bitsra(pC2a_fat, sh), 'like', T.fatigue) + pC2a_sib * cast(W.tj(i3), 'like', T.V), 'like', T.fatigue);
    nC_V   = pC2a_nCV;
    nC_valid = true; nC_idx = pC2a_idx;
  end

  % --- STADIO R (read schedule): programma la lettura del neurone rc ---
  nR_valid = false; nR_idx = uint8(0);
  if rc < uint8(hidden)
    nR_valid = true; nR_idx = rc;
    rc = rc + uint8(1);
  end

  % avanza i registri pipeline (R -> Cm -> Ca -> C1 -> C2 -> write)
  pR_valid = nR_valid; pR_idx = nR_idx;
  pCx_valid = nCx_valid; pCx_idx = nCx_idx; pCx_xsel = nCx_xsel; pCx_Vread = nCx_Vread; pCx_fat = nCx_fat;
  pCm_valid = nCm_valid; pCm_idx = nCm_idx; pCm_Iip = nCm_Iip; pCm_recip = nCm_recip; pCm_Vread = nCm_Vread; pCm_fat = nCm_fat;
  pCa_valid = nCa_valid; pCa_idx = nCa_idx; pCa_reci = nCa_reci; pCa_Ii = nCa_Ii; pCa_Vread = nCa_Vread; pCa_fat = nCa_fat;
  pC1_valid = nC1_valid; pC1_idx = nC1_idx; pC1_Ii = nC1_Ii; pC1_reci = nC1_reci; pC1_Vread = nC1_Vread; pC1_fat = nC1_fat;
  pC2i_valid = nC2i_valid; pC2i_idx = nC2i_idx; pC2i_Vi = nC2i_Vi; pC2i_eth = nC2i_eth; pC2i_fat = nC2i_fat;
  pC2a_valid = nC2a_valid; pC2a_idx = nC2a_idx; pC2a_nCV = nC2a_nCV; pC2a_sib = nC2a_sib; pC2a_fat = nC2a_fat;
  pC_valid = nC_valid; pC_idx = nC_idx; pC_V = nC_V; pC_fat = nC_fat;

  % --- fine tick: tutti i 32 neuroni scritti ---
  if written >= uint8(hidden)
    V_LI = cast(cast(V_LI - bitsra(V_LI, 3), 'like', T.raw) + wacc, 'like', T.raw);
    wacc = cast(zeros(out, 1), 'like', T.raw);
    t_lr = t_lr_nxt;
    t_lr_nxt = cast(zeros(rnk, 1), 'like', T.acc);
    written = uint8(0); rc = uint8(0);
    pR_valid = false; pCx_valid = false; pCm_valid = false; pCa_valid = false; pC1_valid = false; pC2i_valid = false; pC2a_valid = false; pC_valid = false;
    if tickc >= uint8(nt - 1)
      rawreg = V_LI; raw = V_LI; valid = true;
      phase = uint8(0); tickc = uint8(0);
    else
      tickc = tickc + uint8(1);
      xbuf(:, 2:6) = xbuf(:, 1:5); xbuf(:, 1) = xnreg;   % shift+insert per il tick successivo
    end
  end
end

% ---- ROM pesi del champion attivo: in b2_rom_active.m (baked, GENERATO da gen_b2_rom(name)) ----


function p = snn_decode_lut(raw, N) %#codegen
%SNN_DECODE_LUT  Decode Donatello con sigmoide via LUT a N punti su [-8,8) + interp lineare.
%  Generalizza snn_decode_hdl (N=256). N = coder.const, potenza di 2 (scala indice = N/16).
%  Costanti Donatello baked (lo sweep e' Donatello-only). Bit-identico a snn_decode_hdl per N=256.
%
%  ⚠️ SINGLE SOURCE (R4, 2026-07-19): il corpo e' ora la composizione di decode_a + decode_b, che sono
%  le DUE FASI che la chart esegue in due clock distinti -- il decode era il collo (pv_3, 31 livelli:
%  quattro moltiplicatori in serie piu' la lettura di tabella, tutto in un clock).
%  Composte qui in una chiamata sola perche' (a) i chiamanti non cambiano (snn_top_b2, le varianti
%  Donatello_LUT16..512) e (b) i cancelli provano ESATTAMENTE il codice che gira in hardware, non un
%  suo gemello. Il taglio e' fra `frac` e la lettura di `sgtab`: espressioni invariate, solo separate.
  [k, frac] = decode_a(raw, N);
  sv        = decode_b(k, frac, N);
  p         = decode_c(sv);   % [R10] scalatura finale in una fase a se'
end


function [k, frac] = decode_a(raw, N) %#codegen
%DECODE_A  [R4/R12] Prima meta' del decode: dal readout grezzo all'INDICE di tabella + frazione.
%
%  ⚠️ SINGLE SOURCE: composizione di decode_a1 (normalizzazione) e decode_a2 (scala/indice/frazione),
%  che la chart esegue in DUE clock -- i due moltiplicatori erano in serie (collo a 57,5 MHz).
%  Composta qui per i chiamanti funzionali (snn_decode_lut) e perche' i cancelli provino il codice vero.
%
%  ⚠️ NON si time-multiplexano i 5 parametri (restano srotolati): sarebbe un'ottimizzazione di AREA, e
%  di area ce n'e' in abbondanza. Serve solo profondita'.
  adjv        = decode_a1(raw);
  [k, frac]   = decode_a2(adjv, N);
end


function adjv = decode_a1(raw) %#codegen
%DECODE_A1  [R12] Prima parte del decode: normalizzazione (raw - offset)*invtau.
%  Separata da decode_a2 perche' i due moltiplicatori (invtau e scale) erano in serie nello stesso
%  clock -- era il collo a 57,5 MHz (dfrv, 18 livelli). `adj` ha il tipo Tadj GIA' DICHIARATO
%  nell'originale, quindi qui non si stringe nulla (nessun rischio §2.1).
%  Espressione VERBATIM da snn_decode_lut.
  Traw  = numerictype(1,21,13); Tadj = numerictype(1,18,13); Titau = numerictype(1,18,16);
  offset = coder.const(fi([-0.40404 -0.39012 1.7718 2.6884 -0.95578].', Traw));
  invtau = coder.const(fi([0.1 1/3 0.1 1/3 1/3].', Titau));
  adjv = fi(zeros(5,1), Tadj);
  for i = 1:5
    adjv(i) = fi((raw(i) - offset(i)) * invtau(i), Tadj);
  end
end


function [k, frac] = decode_a2(adjv, N) %#codegen
%DECODE_A2  [R12] Seconda parte: scala su [0,N), indice di tabella e frazione.
%  Espressioni VERBATIM da snn_decode_lut, con `adj` gia' calcolato da decode_a1.
  Tadj = numerictype(1,18,13); Ts = numerictype(1,16,14); Tsc = numerictype(0,23,13);
  scale = coder.const(N / 16);                                    % punti per unita' su [-8,8)
  Tsm   = numerictype(0, 8, 0);                                   % moltiplicatore scala (<=32)
  k    = zeros(5, 1, 'int32');
  frac = fi(zeros(5,1), Ts);
  for i = 1:5
    scaled = fi((adjv(i) + fi(8, Tadj)) * fi(scale, Tsm), Tsc);    % (adj+8)*scale in [0,N)
    ki = int32(floor(scaled));
    if ki < int32(0),     ki = int32(0);     end
    if ki > int32(N - 2), ki = int32(N - 2); end
    k(i)    = ki;
    frac(i) = fi(scaled - fi(double(ki), Tsc), Ts);
  end
end


function sv = decode_b(k, frac, N) %#codegen
%DECODE_B  [R4/R10/R17] Seconda fase del decode: tabella + interpolazione lineare -> s.
%  ⚠️ SINGLE SOURCE: composizione di decode_b1 (letture + differenza) e decode_b2 (interpolazione), che
%  la chart esegue in DUE clock. Composta qui per i chiamanti funzionali e per i cancelli.
  [s0v, delv] = decode_b1(k, N);
  sv          = decode_b2(s0v, delv, frac);
end


function [s0v, delv] = decode_b1(k, N) %#codegen
%DECODE_B1  [R17] Letture della tabella + differenza: s0 = sgtab(k), del = sgtab(k+1) - sgtab(k).
%  Separata da decode_b2 perche' letture, sottrazione, moltiplicazione e somma erano tutte nello stesso
%  clock -- era il collo a 77,6 MHz (dsv, 14 livelli). Espressioni VERBATIM da snn_decode_lut.
  Ts    = numerictype(1,16,14);
  scale = coder.const(N / 16);
  sgtab = coder.const(fi(1 ./ (1 + exp(-(-8 + (0:N-1) / scale))), Ts));  % 1xN
  s0v  = fi(zeros(5,1), Ts);
  delv = fi(zeros(5,1), Ts);
  for i = 1:5
    s0 = sgtab(k(i) + 1); s1 = sgtab(k(i) + 2);
    s0v(i)  = s0;
    delv(i) = fi(s1 - s0, Ts);
  end
end


function sv = decode_b2(s0v, delv, frac) %#codegen
%DECODE_B2  [R17] Interpolazione lineare: s = s0 + frac*del. Espressione VERBATIM da snn_decode_lut.
  Ts = numerictype(1,16,14);
  sv = fi(zeros(5,1), Ts);
  for i = 1:5
    sv(i) = fi(s0v(i) + frac(i) * delv(i), Ts);
  end
end


function p = decode_c(sv) %#codegen
%DECODE_C  Scalatura finale -> i 5 parametri. [R10] fase a se' nel controllore.
%  [A3] Ora e' la COMPOSIZIONE di decode_c1 (i prodotti, a precisione piena) + decode_c2 (somma
%  dell'offset + cast). Composta qui perche' (a) i chiamanti non cambiano e (b) i cancelli provano
%  ESATTAMENTE il codice che gira in hardware, non un suo gemello.
%  La chart nella variante `p6` chiama le due meta' in due fasi distinte: e' li' che il taglio serve,
%  perche' separa i DSP dalla catena di CARRY4 che domina il path critico.
  pr = decode_c1(sv);
  p  = decode_c2(pr);
end


function pr = decode_c1(sv) %#codegen
%DECODE_C1  [A3] Prima meta' di decode_c: i SOLI PRODOTTI hilo.*sv.
%  Taglio dentro l'operazione, non fra le operazioni: il collo di Donatello e' `lo + hilo*sv`, dove i
%  DSP fanno la moltiplicazione ma la somma finisce in fabric come catena di 15 CARRY4 in serie
%  (misurato: 24,307 ns = logica 15,490 + routing 8,817, 23 livelli).
%  Registrare il prodotto separa DSP e addizionatore in due clock.
%
%  ⚠️ LARGHEZZA PIENA: il prodotto NON va stretto qui. Stringere un parziale prima dell'uso e' il bug
%  §2.1 di questo progetto — cambierebbe la matematica. Il tipo si lascia DEDURRE dall'espressione.
  Tp   = numerictype(1,21,13);
  hilo = coder.const(fi([37 2 4 2.2 2.5].', Tp));
  pr   = hilo .* sv;                  % tipo dedotto = precisione piena
end


function p = decode_c2(pr) %#codegen
%DECODE_C2  [A3] Seconda meta' di decode_c: somma dell'offset + cast finale ai 5 parametri.
%  Riceve il prodotto a PRECISIONE PIENA da decode_c1 (registrato) e fa `lo + pr`, poi il cast a Q8.13.
%  Aritmetica IDENTICA a decode_c: stesso ordine, stesso singolo cast finale -> bit-exact per
%  costruzione. Ma "per costruzione" non e' un cancello: lo prova run_block_traj_test (dmax=0).
  Tp = numerictype(1,21,13);
  lo = coder.const(fi([8 0.5 1 0.3 0.5].', Tp));
  p  = fi(zeros(5,1), Tp);
  for i = 1:5
    p(i) = fi(lo(i) + pr(i), Tp);
  end
end


function T = acc_types(dt, nfrac, recipN)
%ACC_TYPES  Prototipi di tipo per `acc_iidm_open` type-parametrizzato (modello: snn_types.m).
%  dt = 'double' (riferimento algoritmico + plant cf_plant_lib) | 'fixed' (blocco HDL-ready).
%  nfrac (opz.) = bit frazionari del path fixed; i bit INTERI restano FISSI (il range non cambia),
%  varia solo la risoluzione -> e' la manopola dello sweep (run_acc_fixed_sweep), esattamente come
%  snn_types/run_fixed_sweep fanno per la rete.
%
%  I bit INTERI sono dimensionati con DUE criteri diversi, perche' i limiti hanno natura diversa --
%  applicare a tutti la stessa regola sarebbe misurare la cosa sbagliata:
%
%  (A) limitati dall'OSSERVAZIONE -> margine >= 2x sul massimo misurato (il dataset non e' il mondo).
%      Range misurati su 60 traiettorie x 1000 step coi parametri veri stimati dalla rete (spec SP3 §3):
%    st  : s, v, dv, v_l, s_safe, s_star         max misurato  465.77 -> int 10 (|x|<1024, 2.2x)
%    acc : v_free, a_z, a_iidm, a_cah, a_blend,
%          alf, a_l_bar, dd, z, dv^2/(2*s_safe)  min misurato -288.33 -> int 10 (|x|<1024, 3.6x)
%
%  (B) limitati da un CLAMP -> basta che il tipo copra il limite: non e' una stima, non puo' sforare.
%      Un margine di 1.4x su un limite CERTO vale piu' di 2x su un massimo osservato.
%    par : v0,T,s0,a,b   il decode li vincola a [param_lo, param_hi] = [8 .5 1 .3 .5]..[45 2.5 5 2.5 3]
%                        (sigmoide * range + lo: non puo' uscirne)   -> int  6 (|x|<64, 1.4x su 45)
%    out : accel         il codice la clampa a [-9, a], con a <= 2.5 -> int  4 (|x|<16, 1.8x su 9)
  % nfrac di DEFAULT = 8: il MINIMO che rispetta il budget DERIVATO. Misurato da run_acc_fixed_sweep
  % sul dataset INTERO (60 traj x 1000 step = 60.000 campioni, 2026-07-16, log sweep_nfrac8_60traj.log):
  %   budget  E_snn  (footprint in accel della quantizzazione GIA' accettata della rete):
  %                                   p99 = 0.272054   max = 1.48433  [m/s^2]
  %   nfrac=6 E_iidm  p99 = 0.324937  max = 1.78485  -> NON passa (l'IIDM diventerebbe la fonte
  %                                                     d'errore DOMINANTE, scavalcando la rete)
  %   nfrac=8 E_iidm  p99 = 0.156047  max = 0.83368  -> passa, margine ~1.75x su entrambi
  % ⚠️ Passa STRETTO: un dry-run su 2 traiettorie dava ~6x di margine, il dataset intero dice 1.75x.
  %    Le code stanno solo nel campione completo -> non tarare questo numero su pochi casi.
  if nargin < 2, nfrac = 8; end
  % recipN: strategia di divisione del path fixed. 0 = divide() digit-recurrence (SP3, combinatorio
  % profondo). >0 = reciproco a LUT a recipN punti + moltiplica (SP4 variante L). Vive nei tipi cosi'
  % la scelta e' coder.const e single-source. Default 0 = comportamento SP3 invariato.
  if nargin < 3, recipN = 0; end
  switch dt
    case 'double'
      z = double([]);
      T = struct('st', z, 'par', z, 'acc', z, 'out', z);
      T.recipN = 0;
    case 'fixed'
      f = nfrac;
      % La fimath fa parte del TIPO, non e' una decorazione locale. Due ragioni, entrambe misurate:
      %  1) RoundingMethod 'Zero' e' l'UNICA forma di divisione che HDL Coder genera per tipi signed
      %     ('Floor' vale solo per unsigned, 'Nearest' viene rifiutata) -- spec SP3 §2;
      %  2) attaccarla qui evita che una `setfimath` locale la cambi su una variabile gia' assegnata:
      %     il codegen rifiuta anche il cambio di FIMATH, non solo di tipo -- "Properties of fimath
      %     object must match. Property 'RoundMode' is 'nearest' ... but 'fix'". Mettendola nel
      %     prototipo, ogni cast(x,'like',T.*) la porta con se' e tutto combacia per costruzione.
      % Prodotti e somme a precisione FISSA: senza, i word-length crescerebbero a ogni operazione.
      FM = fimath('RoundingMethod', 'Zero', 'OverflowAction', 'Saturate', ...
                  'ProductMode', 'SpecifyPrecision', ...
                  'ProductWordLength', 11 + f, 'ProductFractionLength', f, ...
                  'SumMode', 'SpecifyPrecision', ...
                  'SumWordLength', 11 + f, 'SumFractionLength', f);
      % Prototipi con valore 0 e NON `fi([])`: un campo VUOTO e' "empty-typed" e HDL Coder lo rifiuta
      % quando lo struct dei tipi attraversa piu' funzioni -- "Struct in expression 'acc_types(''fixed'')'
      % has an empty-typed field. This is not supported for MATLAB-to-dataflow conversion" (SP4-M-FSM:
      % le funzioni-fase iidm_prep/nd/use/final). Come PROTOTIPO e' equivalente: `cast(x,'like',T.*)` usa
      % solo numerictype+fimath, che qui sono identici -> nessun cambiamento numerico (lo provano
      % run_plant_parity, run_block_acciidm_test e G2, tutti ri-eseguiti dopo questa modifica).
      T = struct( ...
        'st',  fi(0, true, 11 + f, f, FM), ...   % Q10.f
        'par', fi(0, true,  7 + f, f, FM), ...   % Q6.f
        'acc', fi(0, true, 11 + f, f, FM), ...   % Q10.f
        'out', fi(0, true,  5 + f, f, FM));      % Q4.f
      T.recipN = recipN;
    otherwise
      error('acc_types:dt', 'dt deve essere ''double'' o ''fixed''');
  end
end


function q = fsm_div(num, den) %#codegen
%FSM_DIV  [SP4-M-FSM] La divisione della forma FSM: UNICA implementazione. FIXED-ONLY.
%  E' la STESSA divisione di acc_div con recipN=0, cioe' SP3: divide(numerictype(T.acc), num, den) con
%  la fimath di acc_types (RoundingMethod 'Zero', l'unica che HDL Coder genera per signed - SP3 §2).
%
%  ⚠️ `T` COSTRUITO DENTRO e non ricevuto come argomento: HDL Coder rifiuta uno struct di prototipi che
%     attraversa le funzioni -- "Struct in expression 'T' has an empty-typed field. This is not supported
%     for MATLAB-to-dataflow conversion" (i prototipi di acc_types sono fi([],...), campi VUOTI).
%     Chiamata qui dentro con argomento letterale, acc_types e' coder.const e viene ripiegata.
%     Conseguenza accettata: la forma FSM e' fixed-only. Il riferimento DOUBLE resta acc_iidm_open
%     (type-parametrico, invariato) -- lo prova run_plant_parity.
%
%  Nella chart del blocco M le 5 divisioni a divisore VARIABILE non passano di qui: sono sostituite
%  dall'handshake verso HDLMathLib/Divide, che G1 ha provato BIT-IDENTICO a questa divide() su 300.000
%  coppie reali (dmax=0). La divisione a divisore COSTANTE (DT del filtro OU) resta qui anche nel blocco:
%  per una costante HDL Coder ripiega un moltiplicatore shallow, non e' un collo di profondita'.
  T = acc_types('fixed');
  q = divide(numerictype(T.acc), num, den);
end


function [st, alf, vlp] = iidm_prep(s, v, dv, v_l, p, rst, alf, vlp, sabin) %#codegen
%IIDM_PREP  [SP4-M-FSM] Fase 0 della FSM: guardie, cast, filtro OU, sab, s_safe -> stato `st`.
%
%  ⚠️ `sabin` (R2, 2026-07-19) = sqrt(af*bf) GIA' CALCOLATA dal chiamante, non piu' qui dentro.
%  Motivo: la radice era il COLLO (17,5 MHz, tutti i 400 path peggiori finivano su st_sab) e per
%  sequenzializzarla serve piu' di un clock -- impossibile dentro una funzione-fase che gira in UNO.
%  Chi chiama la calcola come sa: il model in un colpo (`sqrt_seq`), la chart in 10 stadi con la STESSA
%  ricorrenza (sqrt_seq_step). Vedi iidm_sabx per l'ingresso, che e' a fonte unica.
%  Matematica VERBATIM da acc_iidm_open (righe 24-57): stesse espressioni, stessi cast, stesso ordine.
%
%  UNICA implementazione, chiamata SIA dal model (acc_iidm_fsm, per G2 sul dataset) SIA dalla chart del
%  blocco `Donatello_ACC_IIDM_M` -> la matematica non puo' divergere fra i due (e' il buco §2.1 che
%  costo' l'82,4% dei control-step su snn_b2_fsm: due implementazioni della stessa matematica).
%
%  `st` esce con TUTTI i campi gia' tipizzati (i parziali a zero): da qui in poi i campi non cambiano
%  piu' tipo -- gli aggiornamenti usano `st.campo(:) = ...` (HDL_PHASE §9: una variabile non puo'
%  cambiare ne' tipo ne' fimath).
%
%  ⚠️ Una chiamata per CONTROL-STEP (DT=0.1): il filtro OU stima a_l da Δv_l/DT. Chiamarla a ogni clock
%     farebbe vedere Δv_l=0 per 340 campioni su 341 -> a_l~0, in silenzio (spec SP2 §5).
  % T COSTRUITO DENTRO (non ricevuto): HDL Coder rifiuta uno struct di prototipi che attraversa le
  % funzioni -- "Struct in expression 'T' has an empty-typed field ... MATLAB-to-dataflow conversion"
  % (acc_types usa fi([],...), campi VUOTI). Con argomento letterale e' coder.const -> ripiegata.
%
%  ⚠️ SINGLE SOURCE (R8, 2026-07-19): composizione di iidm_prep_a (SOLO il filtro OU) e
%  iidm_prep_b (cast + costruzione dello struct), che la chart esegue in DUE clock -- il filtro OU
%  era il collo (alf -> a_l_bar, gradini 8 e 9 della scala). G2 prova sui 60000 control-step che il
%  taglio e' bit-neutro.
  [d, alf, vlp] = iidm_prep_a(v_l, rst, alf, vlp);   % R9: differenza finita
  alf           = iidm_prep_a2(d, alf);              % R9: passo esponenziale
  st         = iidm_prep_b(s, v, dv, v_l, p, alf, sabin);
end


function [d, alf, vlp] = iidm_prep_a(v_l, rst, alf, vlp) %#codegen
%IIDM_PREP_A  [R9] Prima meta' del filtro OU: la DIFFERENZA FINITA del leader, d = (lq - vlp)/DT.
%  `d` esce a LARGHEZZA PIENA e senza tipo dichiarato -- lo si lascia dedurre dall'espressione, come per
%  blv in R6: cosi' non si puo' sbagliare la larghezza, e stringerlo cambierebbe la matematica (§2.1).
%
%  ORDINE OBBLIGATO (verbatim da iidm_prep): d usa il vlp VECCHIO, e solo DOPO vlp viene aggiornato.
%  Con rst, vlp = v_l -> d = 0 e alf = 0: inizio traiettoria pulito.
  T = acc_types('fixed');
  DT = 0.1;
  if rst
    alf(:) = 0;
    vlp(:) = v_l;
  end
  lq = cast(v_l, 'like', T.st);
  % Moltiplicazione per 1/DT invece di divide(): vedi iidm_prep. Bit-identita' provata da G2.
  INV_DT = 1/DT;
  d   = (lq - vlp) * INV_DT;
  vlp = cast(lq, 'like', T.st);
end


function alf = iidm_prep_a2(d, alf) %#codegen
%IIDM_PREP_A2  [R9] Seconda meta' del filtro OU: il passo esponenziale.
%  Era il collo a 46,3 MHz (alf_7, 21 livelli): differenza finita e filtro stavano nello stesso clock.
%  Espressione VERBATIM da iidm_prep, con (lq-vlp)*INV_DT gia' calcolato in `d`.
  T = acc_types('fixed');
  DT = 0.1; ALPHA = exp(-DT/1.0);
  alf = cast(ALPHA*alf + (1-ALPHA)*d, 'like', T.acc);
end


function st = iidm_prep_b(s, v, dv, v_l, p, alf, sabin) %#codegen
%IIDM_PREP_B  [R8] Cast, guardie e costruzione dello stato `st`, a partire dall'`alf` GIA' aggiornato
%  da iidm_prep_a (registrato fra i due clock). Espressioni VERBATIM da iidm_prep.
  T = acc_types('fixed');
  v0 = max(p(1), 1e-3); T_ = max(p(2), 1e-3); s0 = p(3);   % a,b -> iidm_ab (servono anche a iidm_sabx)

  sq = cast(s,  'like', T.st);   vq = cast(v,   'like', T.st);
  dq = cast(dv, 'like', T.st);   lq = cast(v_l, 'like', T.st);   %#ok<NASGU>
  v0f = cast(v0, 'like', T.par); Tf_ = cast(T_, 'like', T.par); s0f = cast(s0, 'like', T.par);
  [af, bf] = iidm_ab(p);         % fonte unica, condivisa con iidm_sabx (l'ingresso della radice)

  sab    = cast(max(sabin, 1e-6), 'like', T.par);   % la radice arriva GIA' FATTA
  s_safe = cast(max(sq, 2.0), 'like', T.st);

  % Tipi PIENI dei quadrati (R5/R7): stringerli cambierebbe la matematica (bug §2.1).
  sq0 = cast(0, 'like', T.acc) * cast(0, 'like', T.acc);
  sq1 = sq0 * sq0;
  sq2 = 1 - sq0;
  vt0 = cast(0, 'like', T.st) * cast(0, 'like', T.par);   % [R15] tipo pieno di vq*Tf_     % [R13] tipo pieno di (1 - z^2): isolare la sottrazione dai prodotti

  st = struct( ...
    'vq',      vq, ...
    'dq',      dq, ...
    'v0f',     v0f, ...
    'Tf_',     Tf_, ...
    's0f',     s0f, ...
    'af',      af, ...
    'bf',      bf, ...
    'sab',     sab, ...
    's_safe',  s_safe, ...
    'a_l_bar', cast(min(alf, af), 'like', T.acc), ...
    's_star',  cast(0, 'like', T.st), ...
    'v_free',  cast(0, 'like', T.acc), ...
    'z',       cast(0, 'like', T.acc), ...
    'a_iidm',  cast(0, 'like', T.acc), ...
    'a_cah',   cast(0, 'like', T.acc), ...
    'dd',      cast(0, 'like', T.acc), ...
    'uu',      cast(0, 'like', sq0), ...
    'zz',      cast(0, 'like', sq0), ...
    'uu2',     cast(0, 'like', sq1), ...
    'w',       cast(0, 'like', sq2), ...
    'vt',      cast(0, 'like', vt0), ...
    'qm',      cast(0, 'like', T.acc));
end


function [num, den] = iidm_nd(k, st) %#codegen
%IIDM_ND  [SP4-M-FSM] (num,den) della divisione k, presi dallo stato `st`. UNICA implementazione: la
%  chiamano sia il model (acc_iidm_fsm) sia la chart del blocco M (che li manda al blocco Divide).
%
%  Le 5 divisioni a divisore VARIABILE (ordine = dipendenze: q3 dopo q1 via s_star; q5 dopo q3/q4 via
%  a_iidm/a_cah). Espressioni VERBATIM da acc_iidm_open (righe 56, 58, 59, 68, 70).
%
%  ENTRAMBI in T.acc: il cast e' LOSSLESS (la fimath di acc_types ha Product/SumMode SpecifyPrecision
%  a 11+f bit con f=8 -> ogni prodotto/somma e' GIA' Q10.8 = T.acc; e T.par Q6.8 ⊂ T.acc Q10.8, stessi
%  frazionari). Serve perche' (a) una variabile non puo' cambiare tipo fra i rami (§9) e (b) il blocco
%  Divide ha porte di tipo fisso. G1 ha provato la bit-identita' proprio su coppie in T.acc; G2 ri-verifica
%  end-to-end che il cast non muova un bit.
  T = acc_types('fixed');           % costruito DENTRO (vedi iidm_prep): HDL Coder rifiuta lo struct come arg
  num = cast(0, 'like', T.acc);
  den = cast(1, 'like', T.acc);
  if k == 1                                   % q1 = vq*dq / (2*sab)            -> s_star
    num(:) = st.vq * st.dq;
    den(:) = 2*st.sab;
  elseif k == 2                               % q2 = vq / v0f                   -> v_free
    num(:) = st.vq;
    den(:) = st.v0f;
  elseif k == 3                               % q3 = s_star / s_safe            -> z
    num(:) = st.s_star;
    den(:) = st.s_safe;
  elseif k == 4                               % q4 = max(dq,0)^2 / (2*s_safe)   -> a_cah
    num(:) = max(st.dq, 0)^2;
    den(:) = 2*st.s_safe + 1e-6;
  else                                        % q5 = (a_iidm-a_cah) / bf        -> dd
    num(:) = st.a_iidm - st.a_cah;
    den(:) = st.bf + 1e-6;
  end
end


function st = iidm_use(k, q, st) %#codegen
%IIDM_USE  [SP4-M-FSM] Consuma il quoziente q della divisione k e aggiorna lo stato `st`. UNICA
%  implementazione: la chiamano sia il model (acc_iidm_fsm) sia la chart del blocco M.
%
%  ⚠️ SINGLE SOURCE (R5, 2026-07-19): il corpo e' ora la composizione di iidm_use_a (i quadrati) e
%  iidm_use_b (prodotti e selezioni), che la chart esegue in DUE clock distinti -- k=2 e k=3 erano le
%  due catene piu' profonde della legge (quattro e due moltiplicatori in serie). Composte qui in una
%  chiamata sola: il model resta a un passo e G2 prova sui 60000 control-step che il taglio e' bit-neutro.
  st = iidm_use_a(k, q, st);
  st = iidm_use_m(k, st);      % [R7/R16] primi quadrati
  st = iidm_use_m2(k, st);     % [R16] secondo quadrato / sottrazione
  st = iidm_use_b(k, q, st);
end


function st = iidm_use_a(k, q, st) %#codegen
%IIDM_USE_A  [R5/R16] Prima fase del consumo del quoziente: SOLO i clamp (nessuna moltiplicazione).
%  La legge IIDM ha due catene lunghe, ora distribuite su QUATTRO fasi:
%    k=2  min -> ^2 -> ^2 -> *af      (v_free)
%    k=3  min -> ^2 -> (1-z^2) -> *   (a_iidm)
%  Qui sta solo il primo anello: il clamp. Era il collo a 72,9 MHz (st_uu: min e quadrato insieme).
  if k == 2
    st.qm(:) = min(q, 10);
  elseif k == 3
    st.z(:)  = min(q, 20);
  end
end


function st = iidm_use_m(k, st) %#codegen
%IIDM_USE_M  [R7] Fase di MEZZO del consumo del quoziente: il secondo quadrato di k=2.
%  st.v_free = af*(1 - min(q,10)^4) aveva ANCORA due moltiplicatori in serie dopo R5 (uu^2, poi *af):
%  era il collo a 42,6 MHz (st_v_free, 25 livelli). Qui si isola uu^2 dietro un registro.
%  Il campo `uu2` ha il tipo PIENO (~104 bit): costa registri, non moltiplicatori -- il prodotto
%  esisteva gia', si sta solo mettendo un registro DOPO di esso.
  if k == 1
    st.vt(:) = st.vq * st.Tf_;   % [R15] il prodotto esce dal clock di s_star
  elseif k == 2
    st.uu(:) = st.qm^2;          % [R16] primo quadrato (qm = min(q,10) da iidm_use_a)
  elseif k == 3
    st.zz(:) = st.z^2;           % [R16] quadrato di z
  end
end


function st = iidm_use_m2(k, st) %#codegen
%IIDM_USE_M2  [R16] Terza fase: il secondo quadrato di k=2 e la sottrazione di k=3.
%  Espressioni VERBATIM; i campi hanno il tipo PIENO del prodotto (vedi iidm_prep_b).
  if k == 2
    st.uu2(:) = st.uu^2;
  elseif k == 3
    st.w(:) = 1 - st.zz;
  end
end


function st = iidm_use_b(k, q, st) %#codegen
%IIDM_USE_B  [R5] Seconda meta': i prodotti e le selezioni, a partire dai quadrati gia' registrati.
%  Espressioni VERBATIM da iidm_use, con `min(q,10)^4` -> `st.uu^2` e `st.z^2` -> `st.zz`: identita'
%  garantita solo perche' uu/zz sono a LARGHEZZA PIENA (iidm_prep). Il cancello e' G2 sui 60000
%  control-step -- non si assume che le due forme coincidano, si prova.
  T = acc_types('fixed');
  if k == 1                                   % q1 -> s_star
    st.s_star(:) = st.s0f + max(st.vt + q, 0);   % [R15] vt = vq*Tf_ arriva da iidm_use_m

  elseif k == 2                               % q2 -> v_free
    st.v_free(:) = st.af*(1 - st.uu2);   % [R7] uu2 = uu^2 arriva da iidm_use_m

  elseif k == 3                               % q3 -> a_z / a_iidm (z e z^2 arrivano da iidm_use_a)
    below = (st.vq <= st.v0f);
    a_z = cast(st.af*st.w, 'like', T.acc);
    if st.z < 1
      if below, st.a_iidm(:) = st.v_free*st.w; else, st.a_iidm(:) = st.v_free; end
    else
      if below, st.a_iidm(:) = a_z;                   else, st.a_iidm(:) = st.v_free + a_z; end
    end

  elseif k == 4                               % q4 -> a_cah (+ clamp)
    st.a_cah(:) = st.a_l_bar - q;
    st.a_cah(:) = min(max(st.a_cah, -9), st.af);

  else                                        % q5 -> dd
    st.dd(:) = q;
  end
end


function th = iidm_tanh(st) %#codegen
%IIDM_TANH  [SP4-M-FSM · B2.0-2b] Stadio del tanh: th = tanh(st.dd), via LUT PIENA bit-exact.
%  Dopo lo Studio 2b (document/SP4_ACC_IIDM_FAST.md §Studio 2b): il `tanh` nativo di HDL Coder era il
%  collo combinatorio (198 livelli, 9,42 MHz standalone). `tanh_lut_full` lo MEMOIZZA (LUT 4096 su
%  [-8,8) + 2 costanti di saturazione) -> **dmax=0**, bit-identico al nativo (provato: probe_tanh_dmax
%  = 0 su 20000 control-step a livello accel), ma **8 livelli / 136 MHz standalone e 0 DSP**, ed e' piu'
%  PICCOLA del nativo (545 vs 2190 LUT). Nel controllore intero il tanh non e' piu' il collo (L2 ~10,58,
%  cappato da SNN->decode).
%
%  ⚠️ th resta sfix19_En17 (tipo nativo del tanh): NON castarlo a T.acc (En8) -> butterebbe i bit
%     frazionari prima del prodotto per bf in iidm_final (bug §2.1). La LUT emette gia' sfix19_En17.
%  Confronto delle 5 varianti (native/LUT/interp/poly/CORDIC): SP4_ACC_IIDM_FAST.md §Studio 2b.
%  `tanh_lut_full` e' inlinata nel chart da build_hdl_variants; la tabella la genera gen_tanh_lut().
  th = tanh_lut_full(st.dd);
end


function th = tanh_lut_full(dd) %#codegen
% [B2.0-2b A1] tanh via LUT PIENA bit-exact: memoizza tanh(fi(x,1,19,8)) su [-8,8),
%  saturazione oltre. th: sfix19_En17. GENERATO da gen_tanh_lut.m -- NON modificare a mano.
  persistent TBL
  if isempty(TBL)
    TBL = int32([ ...
      -131070
      -131070
      -131070
      -131070
      -131070
      -131070
      -131070
      -131070
      -131070
      -131070
      -131070
      -131070
      -131070
      -131070
      -131070
      -131070
      -131070
      -131070
      -131070
      -131070
      -131070
      -131070
      -131070
      -131070
      -131070
      -131070
      -131070
      -131070
      -131070
      -131070
      -131070
      -131070
      -131070
      -131070
      -131070
      -131070
      -131070
      -131070
      -131070
      -131070
      -131070
      -131070
      -131070
      -131070
      -131070
      -131070
      -131070
      -131070
      -131070
      -131070
      -131070
      -131070
      -131070
      -131070
      -131070
      -131070
      -131070
      -131070
      -131070
      -131070
      -131070
      -131070
      -131070
      -131070
      -131070
      -131070
      -131070
      -131070
      -131070
      -131070
      -131070
      -131070
      -131070
      -131070
      -131070
      -131070
      -131070
      -131070
      -131070
      -131070
      -131070
      -131070
      -131070
      -131070
      -131070
      -131070
      -131070
      -131070
      -131070
      -131070
      -131070
      -131070
      -131070
      -131070
      -131070
      -131070
      -131070
      -131070
      -131070
      -131070
      -131070
      -131070
      -131070
      -131070
      -131070
      -131070
      -131070
      -131070
      -131070
      -131070
      -131070
      -131070
      -131070
      -131070
      -131070
      -131070
      -131070
      -131070
      -131070
      -131070
      -131070
      -131070
      -131070
      -131070
      -131070
      -131070
      -131070
      -131070
      -131070
      -131070
      -131070
      -131070
      -131070
      -131070
      -131070
      -131070
      -131070
      -131070
      -131070
      -131070
      -131070
      -131070
      -131070
      -131070
      -131070
      -131070
      -131070
      -131070
      -131070
      -131070
      -131070
      -131070
      -131070
      -131070
      -131070
      -131070
      -131070
      -131070
      -131070
      -131070
      -131070
      -131070
      -131070
      -131070
      -131070
      -131070
      -131070
      -131070
      -131070
      -131070
      -131070
      -131070
      -131070
      -131070
      -131070
      -131070
      -131070
      -131070
      -131070
      -131070
      -131070
      -131070
      -131070
      -131070
      -131070
      -131070
      -131070
      -131070
      -131070
      -131070
      -131070
      -131070
      -131070
      -131070
      -131070
      -131070
      -131070
      -131070
      -131070
      -131070
      -131070
      -131070
      -131070
      -131070
      -131070
      -131070
      -131070
      -131070
      -131070
      -131070
      -131070
      -131070
      -131070
      -131070
      -131070
      -131070
      -131070
      -131070
      -131070
      -131070
      -131070
      -131070
      -131070
      -131070
      -131070
      -131070
      -131070
      -131070
      -131070
      -131070
      -131070
      -131070
      -131070
      -131070
      -131070
      -131070
      -131070
      -131070
      -131070
      -131070
      -131070
      -131070
      -131070
      -131070
      -131070
      -131070
      -131070
      -131070
      -131070
      -131070
      -131070
      -131070
      -131070
      -131070
      -131070
      -131070
      -131070
      -131070
      -131070
      -131070
      -131070
      -131070
      -131070
      -131070
      -131070
      -131070
      -131070
      -131070
      -131070
      -131070
      -131070
      -131070
      -131070
      -131070
      -131070
      -131070
      -131070
      -131070
      -131070
      -131070
      -131070
      -131070
      -131070
      -131070
      -131070
      -131070
      -131070
      -131070
      -131070
      -131070
      -131070
      -131070
      -131070
      -131070
      -131070
      -131070
      -131070
      -131070
      -131070
      -131070
      -131070
      -131070
      -131070
      -131070
      -131070
      -131070
      -131070
      -131070
      -131070
      -131070
      -131070
      -131070
      -131070
      -131070
      -131070
      -131070
      -131070
      -131070
      -131070
      -131070
      -131070
      -131070
      -131070
      -131070
      -131070
      -131070
      -131070
      -131070
      -131070
      -131070
      -131070
      -131070
      -131070
      -131070
      -131070
      -131070
      -131070
      -131070
      -131070
      -131070
      -131070
      -131070
      -131070
      -131070
      -131070
      -131070
      -131070
      -131070
      -131070
      -131070
      -131070
      -131070
      -131070
      -131070
      -131070
      -131070
      -131070
      -131070
      -131070
      -131070
      -131070
      -131070
      -131070
      -131070
      -131070
      -131070
      -131070
      -131070
      -131070
      -131070
      -131070
      -131070
      -131070
      -131070
      -131070
      -131070
      -131070
      -131070
      -131070
      -131070
      -131070
      -131070
      -131070
      -131070
      -131070
      -131070
      -131070
      -131070
      -131070
      -131070
      -131070
      -131070
      -131070
      -131070
      -131070
      -131070
      -131070
      -131070
      -131070
      -131070
      -131070
      -131070
      -131070
      -131070
      -131070
      -131070
      -131070
      -131070
      -131070
      -131070
      -131070
      -131070
      -131070
      -131070
      -131070
      -131070
      -131070
      -131070
      -131070
      -131070
      -131070
      -131070
      -131070
      -131070
      -131070
      -131070
      -131070
      -131070
      -131070
      -131070
      -131070
      -131070
      -131070
      -131070
      -131070
      -131070
      -131070
      -131070
      -131070
      -131070
      -131070
      -131070
      -131070
      -131070
      -131070
      -131070
      -131070
      -131070
      -131070
      -131070
      -131070
      -131070
      -131070
      -131070
      -131070
      -131070
      -131070
      -131070
      -131070
      -131070
      -131070
      -131070
      -131070
      -131070
      -131070
      -131070
      -131070
      -131070
      -131070
      -131070
      -131070
      -131070
      -131070
      -131070
      -131070
      -131070
      -131070
      -131070
      -131070
      -131070
      -131070
      -131070
      -131070
      -131070
      -131070
      -131070
      -131070
      -131070
      -131070
      -131070
      -131070
      -131070
      -131070
      -131070
      -131070
      -131070
      -131070
      -131070
      -131070
      -131070
      -131070
      -131070
      -131070
      -131070
      -131070
      -131070
      -131070
      -131070
      -131070
      -131070
      -131070
      -131070
      -131070
      -131070
      -131070
      -131070
      -131070
      -131070
      -131070
      -131070
      -131070
      -131070
      -131070
      -131070
      -131070
      -131070
      -131070
      -131070
      -131070
      -131070
      -131070
      -131070
      -131070
      -131070
      -131070
      -131070
      -131070
      -131070
      -131070
      -131070
      -131070
      -131070
      -131070
      -131070
      -131070
      -131070
      -131070
      -131070
      -131070
      -131070
      -131070
      -131070
      -131070
      -131070
      -131070
      -131070
      -131070
      -131070
      -131070
      -131070
      -131070
      -131070
      -131070
      -131070
      -131070
      -131070
      -131070
      -131070
      -131070
      -131070
      -131070
      -131070
      -131070
      -131070
      -131070
      -131070
      -131070
      -131070
      -131070
      -131070
      -131070
      -131070
      -131070
      -131070
      -131070
      -131070
      -131070
      -131070
      -131070
      -131070
      -131070
      -131070
      -131070
      -131070
      -131070
      -131070
      -131070
      -131070
      -131070
      -131070
      -131070
      -131070
      -131070
      -131070
      -131070
      -131070
      -131070
      -131070
      -131070
      -131070
      -131070
      -131070
      -131070
      -131070
      -131070
      -131070
      -131070
      -131070
      -131070
      -131070
      -131070
      -131070
      -131070
      -131070
      -131070
      -131070
      -131070
      -131070
      -131070
      -131070
      -131070
      -131070
      -131070
      -131070
      -131070
      -131070
      -131070
      -131070
      -131070
      -131070
      -131070
      -131070
      -131070
      -131070
      -131070
      -131070
      -131070
      -131070
      -131070
      -131070
      -131070
      -131070
      -131070
      -131070
      -131070
      -131070
      -131070
      -131070
      -131070
      -131070
      -131070
      -131070
      -131070
      -131070
      -131070
      -131070
      -131070
      -131070
      -131070
      -131070
      -131070
      -131070
      -131070
      -131070
      -131070
      -131070
      -131070
      -131070
      -131070
      -131070
      -131070
      -131070
      -131070
      -131070
      -131070
      -131070
      -131070
      -131070
      -131070
      -131070
      -131070
      -131070
      -131070
      -131070
      -131070
      -131070
      -131070
      -131070
      -131070
      -131070
      -131070
      -131070
      -131070
      -131070
      -131070
      -131070
      -131070
      -131070
      -131070
      -131070
      -131070
      -131070
      -131070
      -131070
      -131070
      -131070
      -131070
      -131070
      -131070
      -131070
      -131070
      -131070
      -131070
      -131070
      -131070
      -131070
      -131070
      -131070
      -131070
      -131070
      -131070
      -131070
      -131070
      -131070
      -131070
      -131070
      -131070
      -131070
      -131070
      -131070
      -131070
      -131070
      -131070
      -131070
      -131070
      -131070
      -131070
      -131070
      -131070
      -131070
      -131070
      -131070
      -131070
      -131070
      -131070
      -131070
      -131070
      -131070
      -131070
      -131070
      -131070
      -131070
      -131070
      -131070
      -131070
      -131070
      -131070
      -131070
      -131062
      -131070
      -131070
      -131070
      -131070
      -131070
      -131070
      -131070
      -131070
      -131070
      -131070
      -131070
      -131070
      -131070
      -131070
      -131070
      -131070
      -131070
      -131070
      -131070
      -131066
      -131070
      -131066
      -131070
      -131058
      -131062
      -131070
      -131070
      -131070
      -131070
      -131070
      -131070
      -131070
      -131070
      -131070
      -131070
      -131070
      -131070
      -131070
      -131070
      -131070
      -131070
      -131070
      -131070
      -131070
      -131070
      -131070
      -131070
      -131070
      -131070
      -131070
      -131070
      -131070
      -131070
      -131070
      -131070
      -131070
      -131070
      -131066
      -131070
      -131070
      -131070
      -131070
      -131070
      -131070
      -131070
      -131070
      -131070
      -131066
      -131070
      -131058
      -131066
      -131058
      -131070
      -131070
      -131070
      -131070
      -131070
      -131070
      -131070
      -131070
      -131066
      -131070
      -131070
      -131070
      -131066
      -131066
      -131070
      -131062
      -131062
      -131066
      -131066
      -131054
      -131070
      -131066
      -131058
      -131066
      -131058
      -131054
      -131046
      -131070
      -131070
      -131070
      -131070
      -131070
      -131058
      -131058
      -131066
      -131058
      -131050
      -131070
      -131066
      -131062
      -131058
      -131066
      -131062
      -131058
      -131062
      -131058
      -131058
      -131058
      -131050
      -131058
      -131054
      -131050
      -131042
      -131058
      -131054
      -131054
      -131046
      -131070
      -131070
      -131070
      -131070
      -131058
      -131058
      -131058
      -131054
      -131070
      -131058
      -131070
      -131070
      -131054
      -131054
      -131054
      -131042
      -131058
      -131070
      -131070
      -131070
      -131042
      -131058
      -131042
      -131054
      -131054
      -131070
      -131042
      -131058
      -131042
      -131054
      -131038
      -131042
      -131042
      -131042
      -131070
      -131054
      -131070
      -131042
      -131038
      -131054
      -131042
      -131058
      -131042
      -131054
      -131058
      -131042
      -131054
      -131042
      -131042
      -131038
      -131058
      -131038
      -131038
      -131058
      -131042
      -131058
      -131038
      -131038
      -131054
      -131042
      -131042
      -131038
      -131038
      -131038
      -131042
      -131054
      -131038
      -131038
      -131042
      -131038
      -131026
      -131026
      -131026
      -131058
      -131042
      -131038
      -131054
      -131054
      -131038
      -131042
      -131042
      -131010
      -131026
      -131026
      -131054
      -131042
      -131026
      -131038
      -131042
      -131010
      -131038
      -131026
      -131026
      -131038
      -131022
      -131010
      -131038
      -131038
      -131022
      -131026
      -131026
      -131006
      -131038
      -131022
      -131010
      -131022
      -131010
      -131006
      -131010
      -131022
      -131006
      -131022
      -131010
      -131006
      -131010
      -131006
      -131006
      -131006
      -131010
      -131006
      -131026
      -131022
      -131038
      -131038
      -131006
      -131006
      -130982
      -130994
      -130990
      -130990
      -130994
      -130994
      -130986
      -130982
      -130994
      -130978
      -130986
      -130978
      -130982
      -130978
      -130986
      -130990
      -130982
      -130978
      -130974
      -130978
      -130978
      -130978
      -130978
      -130978
      -130974
      -130970
      -130974
      -130974
      -130970
      -130966
      -130966
      -130974
      -130974
      -130966
      -130966
      -130974
      -130962
      -130954
      -130962
      -130954
      -130966
      -130962
      -130966
      -130966
      -130958
      -130962
      -130950
      -130958
      -130954
      -130954
      -130954
      -130958
      -130946
      -130946
      -130950
      -130946
      -130946
      -130946
      -130942
      -130942
      -130938
      -130942
      -130942
      -130942
      -130938
      -130926
      -130934
      -130942
      -130938
      -130942
      -130930
      -130934
      -130922
      -130938
      -130934
      -130926
      -130934
      -130934
      -130914
      -130922
      -130918
      -130918
      -130926
      -130918
      -130926
      -130902
      -130902
      -130910
      -130906
      -130910
      -130902
      -130898
      -130898
      -130910
      -130898
      -130894
      -130898
      -130898
      -130890
      -130886
      -130886
      -130898
      -130882
      -130890
      -130882
      -130886
      -130874
      -130878
      -130878
      -130878
      -130870
      -130878
      -130874
      -130874
      -130874
      -130870
      -130870
      -130858
      -130862
      -130850
      -130862
      -130854
      -130858
      -130854
      -130850
      -130842
      -130854
      -130850
      -130850
      -130842
      -130846
      -130830
      -130834
      -130830
      -130830
      -130818
      -130818
      -130818
      -130818
      -130818
      -130818
      -130818
      -130818
      -130818
      -130814
      -130814
      -130818
      -130814
      -130802
      -130814
      -130814
      -130802
      -130802
      -130814
      -130786
      -130786
      -130786
      -130782
      -130782
      -130770
      -130782
      -130766
      -130770
      -130754
      -130770
      -130782
      -130770
      -130754
      -130750
      -130754
      -130754
      -130754
      -130750
      -130750
      -130750
      -130722
      -130734
      -130722
      -130722
      -130722
      -130722
      -130722
      -130722
      -130722
      -130722
      -130690
      -130706
      -130706
      -130718
      -130706
      -130690
      -130690
      -130706
      -130690
      -130686
      -130670
      -130686
      -130670
      -130686
      -130658
      -130658
      -130670
      -130658
      -130654
      -130658
      -130642
      -130654
      -130638
      -130638
      -130638
      -130626
      -130626
      -130622
      -130622
      -130606
      -130622
      -130594
      -130606
      -130606
      -130610
      -130594
      -130574
      -130590
      -130594
      -130562
      -130562
      -130562
      -130562
      -130562
      -130562
      -130562
      -130558
      -130558
      -130558
      -130542
      -130546
      -130546
      -130530
      -130526
      -130546
      -130514
      -130526
      -130498
      -130514
      -130498
      -130494
      -130478
      -130498
      -130466
      -130462
      -130446
      -130462
      -130462
      -130450
      -130450
      -130462
      -130422
      -130430
      -130426
      -130414
      -130414
      -130402
      -130398
      -130398
      -130382
      -130382
      -130382
      -130366
      -130366
      -130354
      -130350
      -130342
      -130342
      -130338
      -130326
      -130330
      -130318
      -130318
      -130306
      -130302
      -130290
      -130290
      -130282
      -130282
      -130274
      -130270
      -130258
      -130250
      -130242
      -130238
      -130230
      -130230
      -130226
      -130210
      -130210
      -130202
      -130202
      -130182
      -130178
      -130174
      -130170
      -130146
      -130146
      -130142
      -130138
      -130114
      -130114
      -130114
      -130094
      -130098
      -130082
      -130082
      -130074
      -130070
      -130050
      -130050
      -130050
      -130046
      -130034
      -130018
      -130014
      -130014
      -129994
      -129994
      -129982
      -129974
      -129958
      -129954
      -129942
      -129934
      -129922
      -129922
      -129914
      -129902
      -129894
      -129878
      -129874
      -129858
      -129858
      -129842
      -129834
      -129826
      -129818
      -129794
      -129790
      -129790
      -129774
      -129770
      -129750
      -129738
      -129738
      -129718
      -129718
      -129706
      -129702
      -129674
      -129662
      -129658
      -129646
      -129634
      -129626
      -129622
      -129598
      -129582
      -129582
      -129558
      -129546
      -129538
      -129534
      -129518
      -129506
      -129490
      -129474
      -129474
      -129462
      -129438
      -129430
      -129418
      -129406
      -129390
      -129378
      -129362
      -129346
      -129334
      -129318
      -129310
      -129298
      -129282
      -129278
      -129262
      -129246
      -129218
      -129214
      -129202
      -129182
      -129154
      -129150
      -129138
      -129122
      -129090
      -129090
      -129086
      -129074
      -129038
      -129026
      -129022
      -129022
      -128990
      -128990
      -128958
      -128942
      -128914
      -128910
      -128898
      -128866
      -128834
      -128834
      -128830
      -128798
      -128782
      -128766
      -128766
      -128734
      -128702
      -128702
      -128670
      -128642
      -128638
      -128622
      -128590
      -128578
      -128546
      -128514
      -128514
      -128510
      -128478
      -128446
      -128446
      -128414
      -128386
      -128370
      -128354
      -128322
      -128318
      -128286
      -128258
      -128242
      -128210
      -128206
      -128190
      -128158
      -128126
      -128098
      -128078
      -128062
      -128034
      -128002
      -127998
      -127970
      -127938
      -127934
      -127902
      -127870
      -127842
      -127822
      -127790
      -127758
      -127742
      -127730
      -127698
      -127650
      -127634
      -127618
      -127570
      -127554
      -127538
      -127490
      -127486
      -127458
      -127406
      -127378
      -127362
      -127342
      -127298
      -127266
      -127234
      -127214
      -127170
      -127154
      -127118
      -127102
      -127038
      -127038
      -126994
      -126974
      -126958
      -126910
      -126898
      -126850
      -126818
      -126786
      -126750
      -126722
      -126702
      -126654
      -126622
      -126574
      -126546
      -126526
      -126462
      -126462
      -126414
      -126354
      -126322
      -126286
      -126254
      -126210
      -126174
      -126138
      -126098
      -126062
      -126022
      -125982
      -125950
      -125906
      -125870
      -125822
      -125786
      -125742
      -125698
      -125666
      -125618
      -125578
      -125534
      -125490
      -125446
      -125410
      -125366
      -125326
      -125270
      -125238
      -125186
      -125142
      -125098
      -125054
      -124998
      -124946
      -124922
      -124866
      -124818
      -124770
      -124726
      -124670
      -124630
      -124574
      -124522
      -124478
      -124418
      -124378
      -124322
      -124270
      -124222
      -124158
      -124114
      -124058
      -124002
      -123946
      -123902
      -123842
      -123782
      -123734
      -123670
      -123622
      -123554
      -123506
      -123438
      -123390
      -123334
      -123266
      -123202
      -123150
      -123094
      -123026
      -122958
      -122902
      -122858
      -122786
      -122726
      -122666
      -122606
      -122530
      -122466
      -122394
      -122350
      -122274
      -122206
      -122138
      -122078
      -121986
      -121922
      -121858
      -121794
      -121726
      -121654
      -121586
      -121506
      -121438
      -121366
      -121286
      -121214
      -121134
      -121062
      -120982
      -120910
      -120834
      -120766
      -120686
      -120606
      -120530
      -120446
      -120358
      -120294
      -120194
      -120118
      -120046
      -119946
      -119866
      -119794
      -119698
      -119622
      -119534
      -119442
      -119354
      -119274
      -119182
      -119094
      -119006
      -118906
      -118810
      -118738
      -118638
      -118538
      -118454
      -118358
      -118270
      -118170
      -118078
      -117978
      -117878
      -117786
      -117694
      -117570
      -117490
      -117378
      -117262
      -117182
      -117070
      -116978
      -116862
      -116750
      -116670
      -116546
      -116434
      -116334
      -116222
      -116098
      -115998
      -115886
      -115774
      -115678
      -115554
      -115426
      -115314
      -115198
      -115074
      -114946
      -114834
      -114722
      -114622
      -114498
      -114382
      -114242
      -114130
      -114014
      -113874
      -113758
      -113630
      -113502
      -113362
      -113234
      -113106
      -112978
      -112834
      -112702
      -112578
      -112450
      -112302
      -112162
      -112034
      -111886
      -111746
      -111618
      -111486
      -111326
      -111182
      -111042
      -110882
      -110738
      -110594
      -110462
      -110318
      -110162
      -110018
      -109854
      -109694
      -109554
      -109390
      -109246
      -109070
      -108926
      -108766
      -108594
      -108446
      -108286
      -108114
      -107954
      -107790
      -107614
      -107454
      -107282
      -107118
      -106930
      -106766
      -106590
      -106430
      -106258
      -106094
      -105918
      -105726
      -105534
      -105358
      -105182
      -104978
      -104802
      -104606
      -104446
      -104242
      -104062
      -103874
      -103678
      -103486
      -103294
      -103102
      -102910
      -102706
      -102498
      -102306
      -102130
      -101890
      -101698
      -101502
      -101298
      -101090
      -100878
      -100674
      -100430
      -100254
      -100034
      -99826
      -99602
      -99382
      -99170
      -98946
      -98726
      -98506
      -98302
      -98062
      -97838
      -97614
      -97378
      -97154
      -96914
      -96690
      -96450
      -96218
      -95986
      -95742
      -95502
      -95262
      -95022
      -94766
      -94526
      -94274
      -94038
      -93790
      -93534
      -93278
      -93030
      -92770
      -92514
      -92258
      -92002
      -91738
      -91486
      -91206
      -90946
      -90686
      -90410
      -90142
      -89878
      -89602
      -89338
      -89070
      -88778
      -88510
      -88222
      -87946
      -87666
      -87370
      -87086
      -86802
      -86526
      -86226
      -85950
      -85646
      -85346
      -85054
      -84754
      -84466
      -84158
      -83862
      -83554
      -83246
      -82942
      -82638
      -82322
      -82014
      -81718
      -81406
      -81086
      -80766
      -80438
      -80126
      -79806
      -79482
      -79146
      -78834
      -78498
      -78170
      -77826
      -77506
      -77178
      -76830
      -76502
      -76158
      -75810
      -75474
      -75134
      -74778
      -74434
      -74094
      -73738
      -73406
      -73050
      -72698
      -72334
      -71978
      -71622
      -71262
      -70894
      -70542
      -70170
      -69802
      -69442
      -69066
      -68698
      -68326
      -67938
      -67570
      -67198
      -66814
      -66434
      -66050
      -65666
      -65298
      -64914
      -64518
      -64130
      -63746
      -63358
      -62974
      -62570
      -62178
      -61770
      -61386
      -60974
      -60574
      -60162
      -59766
      -59362
      -58954
      -58538
      -58134
      -57722
      -57310
      -56894
      -56474
      -56062
      -55634
      -55230
      -54786
      -54366
      -53946
      -53514
      -53102
      -52670
      -52226
      -51794
      -51366
      -50942
      -50494
      -50054
      -49614
      -49174
      -48746
      -48298
      -47870
      -47422
      -46978
      -46530
      -46074
      -45618
      -45170
      -44714
      -44270
      -43818
      -43358
      -42902
      -42438
      -41986
      -41522
      -41058
      -40606
      -40138
      -39678
      -39194
      -38742
      -38274
      -37802
      -37330
      -36862
      -36382
      -35910
      -35442
      -34962
      -34486
      -34022
      -33538
      -33026
      -32586
      -32102
      -31614
      -31126
      -30654
      -30170
      -29694
      -29186
      -28694
      -28222
      -27734
      -27242
      -26754
      -26258
      -25762
      -25282
      -24770
      -24294
      -23790
      -23294
      -22794
      -22310
      -21802
      -21310
      -20814
      -20310
      -19806
      -19314
      -18798
      -18298
      -17802
      -17298
      -16798
      -16302
      -15794
      -15290
      -14778
      -14274
      -13762
      -13254
      -12746
      -12254
      -11746
      -11230
      -10718
      -10214
      -9702
      -9190
      -8682
      -8190
      -7678
      -7166
      -6650
      -6142
      -5626
      -5122
      -4590
      -4094
      -3578
      -3066
      -2550
      -2046
      -1526
      -1022
      -502
      2
      514
      1026
      1538
      2050
      2562
      3074
      3586
      4094
      4610
      5118
      5630
      6142
      6654
      7166
      7678
      8190
      8690
      9206
      9714
      10226
      10730
      11246
      11750
      12270
      12762
      13274
      13778
      14282
      14786
      15298
      15798
      16306
      16798
      17306
      17806
      18314
      18814
      19318
      19822
      20322
      20814
      21314
      21814
      22306
      22802
      23298
      23802
      24298
      24774
      25282
      25774
      26258
      26750
      27250
      27738
      28226
      28710
      29198
      29694
      30170
      30654
      31138
      31618
      32110
      32586
      33054
      33538
      34010
      34494
      34954
      35442
      35918
      36386
      36866
      37334
      37806
      38274
      38746
      39210
      39678
      40146
      40606
      41066
      41530
      41986
      42450
      42910
      43362
      43822
      44274
      44734
      45170
      45630
      46078
      46526
      46974
      47418
      47866
      48306
      48750
      49174
      49622
      50062
      50494
      50938
      51362
      51798
      52226
      52670
      53102
      53518
      53950
      54370
      54790
      55218
      55646
      56062
      56478
      56894
      57314
      57718
      58130
      58538
      58946
      59362
      59770
      60162
      60570
      60978
      61382
      61770
      62166
      62562
      62962
      63358
      63746
      64134
      64518
      64910
      65294
      65666
      66050
      66434
      66818
      67198
      67582
      67950
      68330
      68702
      69070
      69442
      69802
      70174
      70538
      70910
      71262
      71630
      71974
      72334
      72702
      73050
      73406
      73746
      74102
      74450
      74790
      75134
      75482
      75814
      76162
      76498
      76834
      77174
      77506
      77830
      78174
      78502
      78834
      79154
      79482
      79810
      80126
      80438
      80766
      81078
      81402
      81706
      82010
      82318
      82642
      82946
      83254
      83562
      83870
      84162
      84466
      84758
      85054
      85358
      85642
      85946
      86230
      86526
      86806
      87098
      87378
      87670
      87950
      88230
      88514
      88786
      89058
      89338
      89606
      89886
      90154
      90422
      90686
      90958
      91222
      91486
      91746
      92006
      92266
      92526
      92782
      93038
      93290
      93546
      93794
      94046
      94286
      94530
      94782
      95026
      95266
      95506
      95746
      95990
      96222
      96450
      96686
      96918
      97154
      97386
      97610
      97842
      98062
      98298
      98510
      98734
      98954
      99170
      99386
      99606
      99830
      100046
      100254
      100462
      100674
      100882
      101094
      101306
      101506
      101714
      101906
      102118
      102322
      102514
      102714
      102910
      103106
      103302
      103490
      103686
      103874
      104066
      104258
      104446
      104630
      104814
      104994
      105186
      105370
      105542
      105726
      105906
      106082
      106258
      106438
      106602
      106770
      106946
      107118
      107290
      107458
      107622
      107790
      107962
      108118
      108286
      108446
      108606
      108766
      108926
      109082
      109242
      109398
      109554
      109698
      109854
      110014
      110158
      110318
      110462
      110606
      110750
      110898
      111050
      111190
      111330
      111474
      111614
      111754
      111890
      112034
      112170
      112310
      112442
      112578
      112710
      112846
      112982
      113110
      113238
      113370
      113498
      113630
      113750
      113882
      114002
      114130
      114254
      114374
      114498
      114622
      114734
      114854
      114970
      115086
      115202
      115322
      115438
      115554
      115666
      115774
      115890
      115998
      116110
      116222
      116330
      116438
      116546
      116654
      116758
      116866
      116970
      117074
      117178
      117278
      117382
      117486
      117582
      117686
      117778
      117882
      117982
      118078
      118170
      118270
      118362
      118458
      118550
      118642
      118738
      118822
      118918
      119002
      119094
      119186
      119274
      119362
      119446
      119534
      119618
      119706
      119794
      119874
      119954
      120042
      120122
      120206
      120286
      120366
      120446
      120530
      120606
      120682
      120766
      120838
      120910
      120990
      121066
      121138
      121214
      121294
      121362
      121438
      121506
      121586
      121654
      121726
      121794
      121858
      121930
      121998
      122066
      122138
      122206
      122270
      122342
      122402
      122470
      122534
      122602
      122662
      122726
      122790
      122850
      122906
      122970
      123030
      123094
      123154
      123214
      123274
      123330
      123390
      123446
      123506
      123562
      123622
      123674
      123730
      123786
      123842
      123898
      123950
      124006
      124058
      124110
      124162
      124218
      124270
      124322
      124374
      124422
      124474
      124526
      124574
      124622
      124674
      124722
      124770
      124818
      124866
      124910
      124958
      125002
      125054
      125098
      125142
      125186
      125234
      125274
      125322
      125366
      125406
      125446
      125490
      125538
      125574
      125622
      125662
      125702
      125746
      125786
      125826
      125866
      125906
      125950
      125982
      126018
      126062
      126098
      126142
      126174
      126210
      126246
      126286
      126326
      126362
      126402
      126442
      126466
      126502
      126542
      126586
      126610
      126646
      126682
      126718
      126750
      126782
      126814
      126846
      126878
      126910
      126942
      126974
      126994
      127026
      127058
      127094
      127122
      127154
      127186
      127210
      127242
      127274
      127298
      127330
      127362
      127390
      127422
      127450
      127482
      127494
      127522
      127554
      127582
      127614
      127642
      127666
      127694
      127714
      127746
      127762
      127790
      127810
      127842
      127870
      127894
      127918
      127950
      127966
      127994
      128010
      128034
      128062
      128086
      128102
      128126
      128154
      128170
      128198
      128222
      128246
      128262
      128286
      128306
      128322
      128350
      128370
      128386
      128410
      128434
      128454
      128474
      128494
      128510
      128526
      128550
      128574
      128594
      128610
      128630
      128646
      128670
      128682
      128702
      128722
      128746
      128758
      128770
      128794
      128814
      128830
      128846
      128866
      128882
      128898
      128914
      128930
      128950
      128962
      128982
      128998
      129022
      129026
      129042
      129058
      129070
      129086
      129106
      129118
      129138
      129150
      129162
      129178
      129194
      129210
      129218
      129234
      129250
      129266
      129278
      129290
      129310
      129318
      129338
      129350
      129362
      129378
      129390
      129402
      129410
      129426
      129438
      129454
      129462
      129478
      129490
      129506
      129518
      129534
      129538
      129550
      129562
      129570
      129586
      129598
      129606
      129618
      129630
      129642
      129654
      129662
      129670
      129690
      129698
      129710
      129718
      129726
      129738
      129750
      129762
      129774
      129782
      129790
      129798
      129810
      129822
      129830
      129842
      129846
      129858
      129870
      129878
      129890
      129894
      129906
      129918
      129922
      129930
      129942
      129950
      129954
      129966
      129978
      129986
      129998
      130002
      130010
      130018
      130034
      130042
      130046
      130050
      130058
      130066
      130074
      130078
      130086
      130094
      130102
      130110
      130118
      130126
      130134
      130142
      130146
      130154
      130162
      130170
      130178
      130182
      130190
      130194
      130206
      130210
      130214
      130226
      130234
      130238
      130242
      130250
      130258
      130262
      130274
      130274
      130282
      130290
      130294
      130302
      130306
      130310
      130318
      130322
      130330
      130334
      130338
      130346
      130354
      130358
      130366
      130370
      130374
      130382
      130386
      130394
      130394
      130402
      130406
      130410
      130418
      130422
      130430
      130442
      130446
      130446
      130454
      130458
      130458
      130466
      130474
      130478
      130482
      130490
      130494
      130494
      130510
      130510
      130514
      130510
      130518
      130526
      130530
      130530
      130542
      130546
      130542
      130550
      130558
      130562
      130558
      130562
      130562
      130562
      130574
      130574
      130590
      130590
      130590
      130594
      130594
      130606
      130606
      130610
      130610
      130622
      130622
      130622
      130626
      130626
      130626
      130638
      130638
      130642
      130646
      130650
      130654
      130658
      130662
      130666
      130670
      130674
      130678
      130678
      130686
      130686
      130690
      130686
      130690
      130690
      130698
      130698
      130702
      130706
      130706
      130710
      130710
      130718
      130726
      130722
      130726
      130726
      130734
      130734
      130738
      130746
      130750
      130746
      130750
      130750
      130750
      130754
      130762
      130758
      130762
      130766
      130770
      130774
      130770
      130778
      130782
      130782
      130782
      130782
      130790
      130790
      130794
      130794
      130794
      130798
      130798
      130802
      130806
      130810
      130810
      130810
      130814
      130814
      130814
      130818
      130818
      130822
      130822
      130826
      130830
      130822
      130830
      130834
      130834
      130834
      130842
      130842
      130846
      130846
      130850
      130850
      130846
      130850
      130850
      130858
      130854
      130854
      130862
      130862
      130866
      130866
      130870
      130874
      130866
      130874
      130874
      130878
      130878
      130878
      130882
      130882
      130886
      130882
      130886
      130890
      130886
      130894
      130894
      130894
      130898
      130894
      130898
      130898
      130898
      130902
      130906
      130902
      130906
      130906
      130910
      130910
      130910
      130914
      130914
      130914
      130914
      130922
      130922
      130922
      130922
      130926
      130922
      130926
      130926
      130930
      130926
      130934
      130934
      130934
      130938
      130934
      130938
      130938
      130934
      130938
      130938
      130942
      130942
      130946
      130942
      130946
      130946
      130946
      130946
      130946
      130946
      130946
      130946
      130950
      130950
      130954
      130954
      130954
      130958
      130958
      130962
      130958
      130962
      130962
      130962
      130962
      130962
      130962
      130966
      130966
      130966
      130966
      130970
      130970
      130970
      130970
      130978
      130974
      130978
      130974
      130970
      130974
      130974
      130978
      130978
      130978
      130982
      130982
      130978
      130982
      130982
      130982
      130986
      130986
      130986
      130986
      130986
      130986
      130990
      130998
      131006
      130994
      131006
      130994
      130998
      131006
      131010
      131006
      131006
      131006
      131006
      131006
      131010
      131006
      131010
      131006
      131010
      131006
      131010
      131006
      131006
      131022
      131010
      131010
      131010
      131018
      131022
      131018
      131014
      131010
      131010
      131010
      131010
      131010
      131010
      131022
      131018
      131014
      131018
      131022
      131018
      131014
      131026
      131022
      131026
      131022
      131026
      131022
      131026
      131022
      131026
      131030
      131022
      131026
      131030
      131026
      131026
      131030
      131034
      131026
      131030
      131034
      131026
      131034
      131026
      131030
      131034
      131030
      131030
      131034
      131030
      131034
      131030
      131026
      131038
      131034
      131038
      131034
      131038
      131038
      131030
      131038
      131038
      131042
      131038
      131038
      131042
      131038
      131038
      131042
      131038
      131038
      131034
      131042
      131038
      131038
      131042
      131038
      131038
      131046
      131046
      131042
      131042
      131046
      131042
      131046
      131046
      131042
      131050
      131042
      131042
      131042
      131050
      131042
      131050
      131046
      131042
      131046
      131046
      131046
      131050
      131050
      131042
      131046
      131050
      131046
      131054
      131054
      131046
      131046
      131050
      131050
      131054
      131050
      131046
      131054
      131050
      131050
      131054
      131054
      131050
      131050
      131058
      131054
      131058
      131050
      131058
      131054
      131054
      131054
      131054
      131054
      131054
      131054
      131054
      131054
      131054
      131054
      131058
      131054
      131054
      131054
      131054
      131058
      131054
      131062
      131058
      131058
      131058
      131062
      131062
      131054
      131058
      131058
      131058
      131058
      131058
      131062
      131058
      131062
      131058
      131058
      131058
      131058
      131062
      131054
      131058
      131062
      131058
      131062
      131058
      131058
      131058
      131066
      131062
      131058
      131062
      131058
      131062
      131058
      131058
      131058
      131062
      131058
      131062
      131062
      131062
      131062
      131062
      131062
      131062
      131062
      131062
      131062
      131062
      131066
      131062
      131066
      131062
      131062
      131066
      131066
      131062
      131066
      131062
      131066
      131062
      131062
      131066
      131062
      131062
      131066
      131062
      131062
      131066
      131066
      131062
      131066
      131066
      131066
      131066
      131066
      131070
      131066
      131066
      131066
      131066
      131066
      131066
      131070
      131070
      131070
      131066
      131066
      131070
      131070
      131070
      131070
      131070
      131070
      131070
      131070
      131070
      131070
      131070
      131070
      131070
      131070
      131070
      131070
      131070
      131070
      131070
      131070
      131070
      131070
      131070
      131070
      131070
      131070
      131070
      131070
      131070
      131070
      131070
      131070
      131070
      131070
      131070
      131070
      131070
      131070
      131070
      131070
      131070
      131070
      131070
      131070
      131070
      131070
      131070
      131070
      131070
      131070
      131070
      131070
      131070
      131070
      131070
      131070
      131070
      131070
      131070
      131070
      131070
      131070
      131070
      131070
      131070
      131070
      131070
      131070
      131070
      131070
      131070
      131070
      131070
      131070
      131070
      131070
      131070
      131070
      131070
      131070
      131070
      131070
      131070
      131070
      131070
      131070
      131070
      131070
      131070
      131070
      131070
      131070
      131070
      131070
      131070
      131070
      131070
      131070
      131070
      131070
      131070
      131070
      131070
      131070
      131070
      131070
      131070
      131070
      131070
      131070
      131070
      131070
      131070
      131070
      131070
      131070
      131070
      131070
      131070
      131070
      131070
      131070
      131070
      131070
      131070
      131070
      131070
      131070
      131070
      131070
      131070
      131070
      131070
      131070
      131070
      131070
      131070
      131070
      131070
      131070
      131070
      131070
      131070
      131070
      131070
      131070
      131070
      131070
      131070
      131070
      131070
      131070
      131070
      131070
      131070
      131070
      131070
      131070
      131070
      131070
      131070
      131070
      131070
      131070
      131070
      131070
      131070
      131070
      131070
      131070
      131070
      131070
      131070
      131070
      131070
      131070
      131070
      131070
      131070
      131070
      131070
      131070
      131070
      131070
      131070
      131070
      131070
      131070
      131070
      131070
      131070
      131070
      131070
      131070
      131070
      131070
      131070
      131070
      131070
      131070
      131070
      131070
      131070
      131070
      131070
      131070
      131070
      131070
      131070
      131070
      131070
      131070
      131070
      131070
      131070
      131070
      131070
      131070
      131070
      131070
      131070
      131070
      131070
      131070
      131070
      131070
      131070
      131070
      131070
      131070
      131070
      131070
      131070
      131070
      131070
      131070
      131070
      131070
      131070
      131070
      131070
      131070
      131070
      131070
      131070
      131070
      131070
      131070
      131070
      131070
      131070
      131070
      131070
      131070
      131070
      131070
      131070
      131070
      131070
      131070
      131070
      131070
      131070
      131070
      131070
      131070
      131070
      131070
      131070
      131070
      131070
      131070
      131070
      131070
      131070
      131070
      131070
      131070
      131070
      131070
      131070
      131070
      131070
      131070
      131070
      131070
      131070
      131070
      131070
      131070
      131070
      131070
      131070
      131070
      131070
      131070
      131070
      131070
      131070
      131070
      131070
      131070
      131070
      131070
      131070
      131070
      131070
      131070
      131070
      131070
      131070
      131070
      131070
      131070
      131070
      131070
      131070
      131070
      131070
      131070
      131070
      131070
      131070
      131070
      131070
      131070
      131070
      131070
      131070
      131070
      131070
      131070
      131070
      131070
      131070
      131070
      131070
      131070
      131070
      131070
      131070
      131070
      131070
      131070
      131070
      131070
      131070
      131070
      131070
      131070
      131070
      131070
      131070
      131070
      131070
      131070
      131070
      131070
      131070
      131070
      131070
      131070
      131070
      131070
      131070
      131070
      131070
      131070
      131070
      131070
      131070
      131070
      131070
      131070
      131070
      131070
      131070
      131070
      131070
      131070
      131070
      131070
      131070
      131070
      131070
      131070
      131070
      131070
      131070
      131070
      131070
      131070
      131070
      131070
      131070
      131070
      131070
      131070
      131070
      131070
      131070
      131070
      131070
      131070
      131070
      131070
      131070
      131070
      131070
      131070
      131070
      131070
      131070
      131070
      131070
      131070
      131070
      131070
      131070
      131070
      131070
      131070
      131070
      131070
      131070
      131070
      131070
      131070
      131070
      131070
      131070
      131070
      131070
      131070
      131070
      131070
      131070
      131070
      131070
      131070
      131070
      131070
      131070
      131070
      131070
      131070
      131070
      131070
      131070
      131070
      131070
      131070
      131070
      131070
      131070
      131070
      131070
      131070
      131070
      131070
      131070
      131070
      131070
      131070
      131070
      131070
      131070
      131070
      131070
      131070
      131070
      131070
      131070
      131070
      131070
      131070
      131070
      131070
      131070
      131070
      131070
      131070
      131070
      131070
      131070
      131070
      131070
      131070
      131070
      131070
      131070
      131070
      131070
      131070
      131070
      131070
      131070
      131070
      131070
      131070
      131070
      131070
      131070
      131070
      131070
      131070
      131070
      131070
      131070
      131070
      131070
      131070
      131070
      131070
      131070
      131070
      131070
      131070
      131070
      131070
      131070
      131070
      131070
      131070
      131070
      131070
      131070
      131070
      131070
      131070
      131070
      131070
      131070
      131070
      131070
      131070
      131070
      131070
      131070
      131070
      131070
      131070
      131070
      131070
      131070
      131070
      131070
      131070
      131070
      131070
      131070
      131070
      131070
      131070
      131070
      131070
      131070
      131070
      131070
      131070
      131070
      131070
      131070
      131070
      131070
      131070
      131070
      131070
      131070
      131070
      131070
      131070
      131070
      131070
      131070
      131070
      131070
      131070
      131070
      131070
      131070
      131070
      131070
      131070
      131070
      131070
      131070
      131070
      131070
      131070
      131070
      131070
      131070
      131070
      131070
      131070
      131070
      131070
      131070
      131070
      131070
      131070
      131070
      131070
      131070
      131070
      131070
      131070
      131070
      131070
      131070
      131070
      131070
      131070
      131070
      131070
      131070
      131070
      131070
      131070
      131070
      131070
      131070
      131070
      131070
      131070
      131070
      131070
      131070
      131070
      131070
      131070
      131070
      131070
      131070
      131070
      131070
      131070
      131070
      131070
      131070
      131070
      131070
      131070
      131070
      131070
      131070
      131070
      131070
      131070
      131070
      131070
      131070
      131070
      131070
      131070
      131070
      131070
      131070
      131070
      131070
      131070
      131070
      131070
      131070
      131070
      131070
      131070
      131070
      131070
      131070
      131070
      131070
      131070
      131070
      131070
      131070
      131070
      131070
      131070
      131070
      131070
      131070
      131070
      131070
      131070
      131070
      131070
      131070
      131070
      131070
      131070
      131070
      131070
      131070
      131070
      131070
      131070
      131070
      131070
      131070
      131070
      131070
      131070
      131070
      131070
      131070
      131070
      131070
      131070
      131070
      131070
      131070
      131070
      131070
      131070
      131070
      131070
      131070
      131070
      131070
      131070
      131070
      131070
      131070
      131070
      131070
      131070
      131070
      131070
      131070
      131070
      131070
      131070
      131070
      131070
      131070
      131070
      131070
      131070
      131070
      131070
      131070
      131070
      131070
      131070
      131070
      131070
      131070
      131070
      131070
      131070
      131070
      131070
      131070
      131070
      131070
      131070
      131070
      131070
      131070
      131070
      131070
      131070
      131070
      131070
      131070
      131070
    ]);
  end
  si = int32(storedInteger(dd));
  if si < int32(-2048)
    a = int32(1);
  elseif si > int32(2047)
    a = int32(4096);
  else
    a = si + int32(2049);
  end
  th = reinterpretcast(fi(TBL(a), 1, 19, 0), numerictype(1,19,17));
end


function accel = iidm_final(st, th) %#codegen
%IIDM_FINAL  [SP4-M-FSM] Fase finale: blend ACC + clamp -> accel. UNICA implementazione: la chiamano sia
%  il model (acc_iidm_fsm) sia la chart del blocco M (stato FINAL, dopo lo stato TANH).
%  Espressioni VERBATIM da acc_iidm_open (righe 71-73), con `tanh(st.dd)` che arriva gia' calcolato in
%  `th` da iidm_tanh: e' uno stadio a se' perche' il tanh fixed era il path critico (237 livelli, 7,35).
%  `th` mantiene il suo TIPO NATIVO (nessun cast a T.acc: butterebbe i bit frazionari prima del prodotto
%  con bf -> bug §2.1).
%
%  ⚠️ SINGLE SOURCE (R6, 2026-07-19): composizione di iidm_final_a (a_cah + bf*th) e iidm_final_b
%  (blend + clamp), che la chart esegue in due clock -- `acc` era il collo (35 livelli, due
%  moltiplicatori in serie). G2 prova sui 60000 control-step che il taglio e' bit-neutro.
  accel = iidm_final_c(st, iidm_final_b(st, iidm_final_a(st, th)));   % R11: cast/select/clamp a se'
end


function bl = iidm_final_a(st, th) %#codegen
%IIDM_FINAL_A  [R6] Prima meta' della fase finale: il termine CAH + il prodotto col tanh.
%  bl = a_cah + bf*th, a LARGHEZZA PIENA: e' il valore che attraversa il registro fra le due fasi, e
%  stringerlo qui cambierebbe la matematica (bug §2.1). Il tipo NON si dichiara: lo si lascia dedurre
%  dall'espressione, e la chart lo cattura inizializzando il suo stato con questa stessa funzione.
  bl = st.a_cah + st.bf * th;
end


function ab = iidm_final_b(st, bl) %#codegen
%IIDM_FINAL_B  [R6/R11] Seconda fase della finale: il blend esponenziale ACC, a LARGHEZZA PIENA.
%  Il cast a T.acc, la selezione e il clamp stanno in iidm_final_c: erano tutti nello stesso clock.
%  `ab` non ha tipo dichiarato -- lo si lascia dedurre dall'espressione (come blv in R6), cosi' non si
%  puo' sbagliare la larghezza e non si stringe nulla prima dell'uso (§2.1).
%  Espressione VERBATIM da iidm_final.
  COOL = 0.99;
  ab = (1-COOL)*st.a_iidm + COOL*bl;
end


function accel = iidm_final_c(st, ab) %#codegen
%IIDM_FINAL_C  [R11] Terza fase della finale: cast, selezione ACC e clamp -> accel.
%  Separata da iidm_final_b perche' il blend moltiplicativo e questa catena stavano nello stesso clock
%  (acc_3, 24 livelli, il collo a 52,3 MHz). Espressioni VERBATIM da iidm_final.
  T = acc_types('fixed');
  a_blend = cast(ab, 'like', T.acc);
  if st.a_iidm >= st.a_cah, ac = st.a_iidm; else, ac = a_blend; end
  accel = cast(min(max(ac, -9), st.af), 'like', T.out);
end


function nb = div_seq_nb() %#codegen
%DIV_SEQ_NB  Numero di bit di quoziente della ricorrenza (= cicli dello stadio DIV in HW).
%  T.acc = fixdt(1,19,8): il dividendo scalato e' |N|<<8 con |N| <= 2^18, quindi <= 2^26 -> 27 bit.
%  Costante condivisa fra `div_seq` (wrapper funzionale, provato) e la chart (stessa ricorrenza a stadi):
%  se cambia il tipo, cambia QUI e in un posto solo.
  nb = 27;
end


function [A, B, sq] = div_seq_setup(num, den) %#codegen
%DIV_SEQ_SETUP  [IIDM #2] Preparazione della ricorrenza: magnitudini + segno del quoziente.
%  SINGLE SOURCE con la chart (stadio DIV-INIT) e col wrapper provato `div_seq`.
%
%  ⚠️ NIENTE abs() di fi: abs() SATURA sul valore piu' negativo (-2^(WL-1) -> 2^(WL-1)-1), cioe' sbaglia
%     di 1 LSB proprio sull'estremo. Si passa per l'intero memorizzato in un tipo piu' LARGO, dove la
%     negazione non satura.
  T  = acc_types('fixed');
  nt = numerictype(T.acc);
  WL = nt.WordLength;                 % 19
  FL = nt.FractionLength;             % 8
  NB = div_seq_nb();                  % 27
  NR = 20;

  sq = (num < 0) ~= (den < 0);        % segno del quoziente

  sn = reinterpretcast(num, numerictype(1, WL, 0));      % intero memorizzato, sfix(WL)
  sd = reinterpretcast(den, numerictype(1, WL, 0));
  wn = cast(sn, 'like', fi(0, 1, WL+1, 0));              % sfix(WL+1): -(-2^(WL-1)) ci sta
  wd = cast(sd, 'like', fi(0, 1, WL+1, 0));
  if wn < 0, wn(:) = -wn; end                            % magnitudine, senza saturare
  if wd < 0, wd(:) = -wd; end

  A = bitsll(cast(wn, 'like', fi(0, 0, NB, 0)), FL);     % |N| << FL  (<= 2^26, sta in ufix27)
  B = cast(wd, 'like', fi(0, 0, NR, 0));                 % |D|
end


function [An, Rn, Qn] = div_seq_step(A, R, Q, B) %#codegen
%DIV_SEQ_STEP  [IIDM #2] UN passo della ricorrenza restoring: produce UN bit di quoziente.
%  SINGLE SOURCE: questa identica funzione e' chiamata (a) dalla chart, una volta per ciclo, nello stadio
%  DIV, e (b) dal wrapper funzionale `div_seq`, iterata nb volte, che il cancello prova su 300k coppie
%  REALI. Cosi' cio' che e' PROVATO e' esattamente cio' che GIRA in hardware (stesso principio delle
%  funzioni-fase iidm_*): non esistono due esemplari dell'algoritmo che possano divergere in silenzio.
%
%  Formulazione scelta per l'HW: si consuma A dal MSB e si spinge in R, invece di indicizzare il bit
%  i-esimo. Cosi' gli shift sono FISSI (cablaggio, non muxaggio) e non serve alcun indice variabile --
%  che in HDL diventerebbe un mux a nb vie su ogni passo.
%
%    A : dividendo residuo (consumato dal MSB)   ufix(NB)
%    R : resto parziale                          ufix(NR)
%    Q : quoziente parziale                      ufix(NB)
%    B : divisore (magnitudine)                  ufix(NR)
  abit = bitget(A, div_seq_nb());        % MSB di A (indice FISSO)
  An   = bitsll(A, 1);                   % A <<= 1  (il bit consumato esce)

  Rs = bitsll(R, 1);                     % R <<= 1
  Rs(:) = Rs + cast(abit, 'like', R);    % R = (R << 1) | abit   -- (:) per non cambiare il tipo

  Qs = bitsll(Q, 1);                     % Q <<= 1
  if Rs >= B                             % restoring: sottrai solo se ci sta
    Rn = Rs; Rn(:) = Rs - B;
    Qn = Qs; Qn(:) = Qs + 1;             % ...e il bit di quoziente vale 1
  else
    Rn = Rs;
    Qn = Qs;
  end
end


function q = div_seq_fin(Q, sq, den_is_zero, num_sign) %#codegen
%DIV_SEQ_FIN  [IIDM #2] Finalizzazione: applica il segno al quoziente e satura al range di T.acc.
%  SINGLE SOURCE con la chart (stadio DIV-FIN) e col wrapper provato `div_seq`.
%  den_is_zero/num_sign gestiscono la guardia den=0 (che il controllore non produce -- iidm_prep guarda
%  i denominatori -- ma la funzione non deve esplodere).
  T  = acc_types('fixed');
  nt = numerictype(T.acc);
  WL = nt.WordLength;
  NB = div_seq_nb();

  qw = cast(Q, 'like', fi(0, 1, NB+1, 0));      % sfix(NB+1): ospita il segno senza saturare
  if sq, qw(:) = -qw; end

  if den_is_zero                                 % saturazione al segno del dividendo
    if num_sign > 0
      qw(:) = 2^(WL-1) - 1;
    elseif num_sign < 0
      qw(:) = -2^(WL-1);
    else
      qw(:) = 0;
    end
  end

  qs = fi(qw, 1, WL, 0, fimath('OverflowAction','Saturate','RoundingMethod','Zero'));  % satura a T.acc
  q  = reinterpretcast(removefimath(qs), nt);
end


function nb = sqrt_seq_nb() %#codegen
%SQRT_SEQ_NB  Bit di risultato della radice (= cicli dello stadio SQRT in HW).
%  Ingresso af*bf = numerictype(1,19,8) -> intero memorizzato fino a 2^18-1; la radice intera sta in
%  9 bit (max 511), e servono 10 iterazioni (2 bit di radicando ciascuna, 20 >= 19).
  nb = 10;
end


function X = sqrt_seq_setup(x) %#codegen
%SQRT_SEQ_SETUP  [IIDM R2] Il radicando come intero senza segno: e' lo stato iniziale della ricorrenza.
%
%  Il trucco che regge tutto: FL_out = FL_in/2 esattamente (4 = 8/2), quindi
%      y_stored = floor(sqrt(x_val) * 2^FL_out) = floor(sqrt(X_stored))
%  cioe' basta la RADICE INTERA dell'intero memorizzato -- nessuna riscalatura.
%
%  `reinterpretcast` e non `double(storedInteger(x))`: e' la stessa operazione sui bit, ma sintetizzabile
%  (un rinominare fili, zero hardware) invece di un passaggio in virgola mobile che HDL Coder rifiuta.
%
%  ⚠️ Presuppone x >= 0, ed e' GARANTITO PER COSTRUZIONE, non sperato: af,bf = cast(max(p,1e-3),..) con
%  troncamento verso zero -> af,bf >= 0 -> x = af*bf >= 0. (Il dominio della prova esaustiva e'
%  esattamente questo: 0 .. 1023,996.)
  X = fi(0, 0, sqrt_seq_nb() * 2, 0);
  X(:) = reinterpretcast(x, numerictype(0, 19, 0));
end


function [Xn, Rn, Qn] = sqrt_seq_step(X, R, Q) %#codegen
%SQRT_SEQ_STEP  [IIDM R2] UN passo della radice quadrata digit-recurrence (restoring): produce UN bit.
%  SINGLE SOURCE: identica funzione chiamata (a) dalla chart una volta per ciclo nello stadio SQRT-STEP
%  e (b) dal wrapper `sqrt_seq`, iterata, che il cancello prova su TUTTO il dominio d'ingresso.
%
%  Ricorrenza classica: si consumano DUE bit del radicando per ogni bit di risultato, e si confronta col
%  "quadrato di prova" 4Q+1 -- e' esattamente cio' che HDL Coder chiama `ytempSquare` nel netlist.
%  Shift FISSI (cablaggio, non mux): niente indice variabile.
  two = bitsliceget(X, sqrt_seq_nb()*2, sqrt_seq_nb()*2 - 1);   % i 2 bit piu' alti di X
  Xn  = bitsll(X, 2);                                           % X <<= 2

  Rs = bitsll(R, 2);
  Rs(:) = Rs + cast(two, 'like', R);        % R = (R << 2) | due bit

  tr = bitsll(cast(Q, 'like', R), 2);
  tr(:) = tr + 1;                            % quadrato di prova: 4Q + 1

  Qs = bitsll(Q, 1);
  if Rs >= tr
    Rn = Rs; Rn(:) = Rs - tr;
    Qn = Qs; Qn(:) = Qs + 1;
  else
    Rn = Rs;
    Qn = Qs;
  end
end


function y = sqrt_seq_fin(Q) %#codegen
%SQRT_SEQ_FIN  [IIDM R2] La radice parziale diventa il risultato tipizzato: ufix(10,0) -> sfix(10,4).
%
%  Due `reinterpretcast` in fila, entrambi a costo zero in hardware (rinominano fili):
%    1) ufix(10,0) -> sfix(10,0): lecito perche' Q <= 511 SEMPRE. Q e' la radice intera di un numero a
%       19 bit, quindi Q <= floor(sqrt(2^19-1)) = 724... ma il radicando reale arriva a 262143, da cui
%       Q <= 511 < 2^9: il bit di segno non si accende mai.
%    2) sfix(10,0) -> sfix(10,4): riposiziona la virgola. E' il passo che realizza FL_out = FL_in/2.
  y = reinterpretcast(reinterpretcast(Q, numerictype(1, 10, 0)), numerictype(1, 10, 4));
end


function [af, bf] = iidm_ab(p) %#codegen
%IIDM_AB  [R2] I due parametri di accelerazione/decelerazione tipizzati. Estratti da iidm_prep perche'
%  ORA SERVONO A DUE CHIAMANTI: iidm_prep (che li mette nello struct) e iidm_sabx (che ne fa il
%  prodotto, ingresso della radice sequenziale).
%
%  ⚠️ Esistono per NON duplicare due righe di cast. Sembrano innocue -- `cast(max(p(4),1e-3),'like',T.par)`
%  copiata in due punti "e' ovviamente identica" -- ma e' esattamente la forma del buco §2.1 che costo'
%  l'82,4% dei control-step: due esemplari della stessa matematica che divergono in silenzio.
  T  = acc_types('fixed');
  af = cast(max(p(4), 1e-3), 'like', T.par);
  bf = cast(max(p(5), 1e-3), 'like', T.par);
end


function x = iidm_sabx(p) %#codegen
%IIDM_SABX  [R2] L'INGRESSO della radice: x = af*bf, da cui sab = sqrt(x).
%  Chiamata dal model (che poi fa sqrt_seq(x) in una volta) e dalla chart (che avvia su x la ricorrenza
%  sequenziale, uno stadio per clock). Una sola definizione di "cosa entra nella radice".
  [af, bf] = iidm_ab(p);
  x = iidm_sabx_mul(af, bf);   % [R14] il prodotto e' una funzione a se': la chart lo fa in un clock proprio
end


function x = iidm_sabx_mul(af, bf) %#codegen
%IIDM_SABX_MUL  [R14] Il solo PRODOTTO af*bf, ingresso della radice.
%  Separato dai cast di iidm_ab perche' max/cast e moltiplicazione erano nello stesso clock -- era il
%  collo a 65,3 MHz (sX, 21 livelli). Fonte unica: la usano sia iidm_sabx (per il model) sia la chart.
  x = af * bf;
end
